simulink model "rfi_detection"  (R2013b)
settings: Solver=ode45  StartTime=0.0  StopTime=10.0  RelTol=1e-3
undefined symbols (not defined in the file or in its folder): calan_lib, comp_addsub
libraries: xbsIndex_r4 x2633, casper_library_misc x66, dspsigops x32, simulink x4, casper_library_delays x4, xps_library x2
(part 1 of 22)
settings Model: Creator=root  LastModifiedBy=root
settings DebuggingCC: StateNameClashWarn=warning

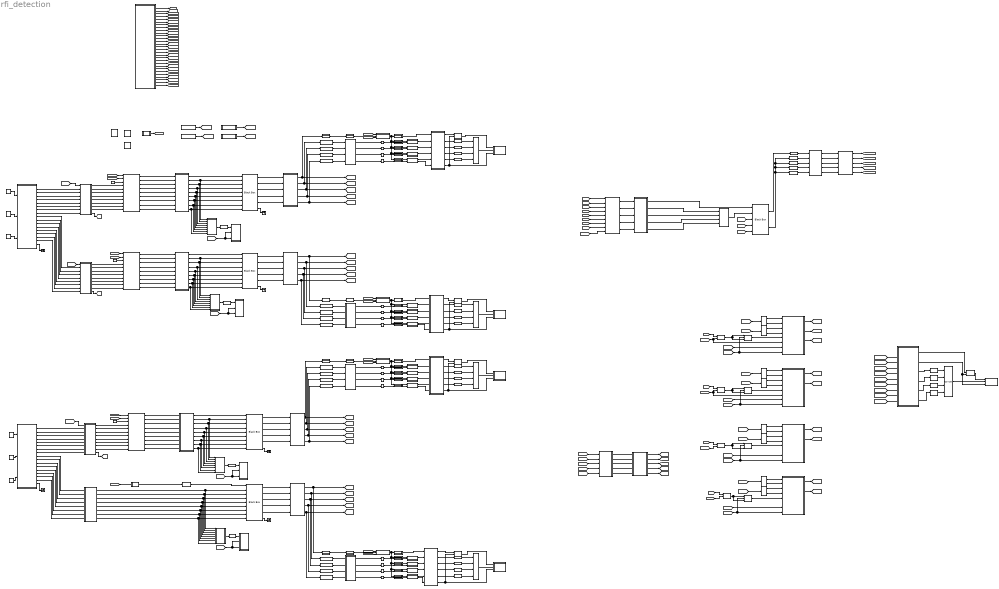
== system rfi_detection ==
  note: TODO!!!
  note: check if we could
      | hardcode the gain
  note: To catch the prog delay
  " System Generator" : xbsIndex_r4/ System Generator  Tag=genX  xilinxfamily=virtex6  part=xc6vsx475t  speed=-1  package=ff1759  synthesis_tool=XST  clock_wrapper=Clock Enables  directory=./arte/sysgen  proj_type=Project Navigator  Synth_file=XST Defaults  Impl_file=ISE Defaults  testbench=off  simulink_period=1  sysclk_period=6.6667  dcm_input_clock_period=100  incr_netlist=off  trim_vbits=Everywhere in SubSystem  dbl_ovrd=According to Block Masks  core_generation=According to Block Masks  run_coregen=off  deprecated_control=off  eval_field=0  block_type=sysgen
  Band-Limited White Noise{,1..3} (4 alike) : simulink/Sources/Band-Limited White Noise  Cov=[0.1]  Ts=0.1  seed=[23341]
  Black Box{1..3,6} (4 alike) : xbsIndex_r4/Black Box  init_code=pfb_fft_8in_2048ch_config  sim_method=Inactive  verbose=off  block_type=blackbox2
  Black Box5 : xbsIndex_r4/Black Box  init_code=fft_channel_flag_top_config  sim_method=Inactive  verbose=off  block_type=blackbox2
  Concat{,1..3,11} (5 alike) : xbsIndex_r4/Concat  num_inputs=4  dbl_ovrd=off  block_type=concat
  Constant11 : xbsIndex_r4/Constant  const=1  gui_display_data_type=Boolean  arith_type=Boolean  n_bits=16  bin_pt=14  preci_type=Single  exp_width=8  frac_width=24  explicit_period=on  period=1  equ=P=C  opselect=C  inp2=PCIN>>17  opr=+  inp1=P  carry=CIN  dbl_ovrd=off  block_type=constant
  Constant13 : Constant
  Constant2 : Constant
  Constant8 : xbsIndex_r4/Constant  const=1  gui_display_data_type=Boolean  arith_type=Boolean  n_bits=16  bin_pt=14  preci_type=Single  exp_width=8  frac_width=24  explicit_period=on  period=1  equ=P=C  opselect=C  inp2=PCIN>>17  opr=+  inp1=P  carry=CIN  dbl_ovrd=off  block_type=constant
  Constant9 : xbsIndex_r4/Constant  const=1  gui_display_data_type=Boolean  arith_type=Boolean  n_bits=16  bin_pt=14  preci_type=Single  exp_width=8  frac_width=24  explicit_period=on  period=1  equ=P=C  opselect=C  inp2=PCIN>>17  opr=+  inp1=P  carry=CIN  dbl_ovrd=off  block_type=constant
  Convert5 : xbsIndex_r4/Convert  gui_display_data_type=Boolean  arith_type=Boolean  n_bits=3  bin_pt=0  float_type=Single  exp_bits=8  fraction_bits=24  quantization=Truncate  overflow=Wrap  en=off  latency=0  dbl_ovrd=off  pipeline=off  block_type=convert
      settings: block_version=11.4
  Counter{1..4,10} (5 alike) : xbsIndex_r4/Counter  cnt_type=Free Running  cnt_to=Inf  operation=Up  start_count=0  cnt_by_val=1  arith_type=Unsigned  n_bits=9  bin_pt=0  load_pin=off  rst=on  en=on  explicit_period=on  period=1  dbl_ovrd=off  use_behavioral_HDL=off  implementation=Fabric  block_type=counter
  Delay{1,7..10,32,34..36,43,45..47,50..52} (16 alike) : xbsIndex_r4/Delay  rst=off  infoeditControl=Selection of Reset will increase slice count due to use of real FFs and instead of SRLs  en=off  latency=1  dbl_ovrd=off  reg_retiming=off  block_type=delay
  Logical{,1..3} (4 alike) : xbsIndex_r4/Logical  logical_function=AND  inputs=2  en=off  latency=0  precision=Full  arith_type=Unsigned  n_bits=16  bin_pt=0  align_bp=on  dbl_ovrd=off  block_type=logical
  Register{,1..3} (4 alike) : xbsIndex_r4/Register  init=0  rst=on  en=on  dbl_ovrd=off  block_type=register
  Reinterpret{1..12,21..26,28,31} (20 alike) : xbsIndex_r4/Reinterpret  force_arith_type=on  arith_type=Unsigned  force_bin_pt=on  bin_pt=0  block_type=reinterpret
  Slice1 : xbsIndex_r4/Slice  nbits=36  boolean_output=off  mode=Lower Bit Location + Width  bit1=0  base1=MSB of Input  bit0=72  base0=LSB of Input  dbl_ovrd=off  block_type=slice
  Slice2 : xbsIndex_r4/Slice  nbits=36  boolean_output=off  mode=Lower Bit Location + Width  bit1=0  base1=MSB of Input  bit0=108  base0=LSB of Input  dbl_ovrd=off  block_type=slice
  Slice3 : xbsIndex_r4/Slice  nbits=36  boolean_output=off  mode=Lower Bit Location + Width  bit1=0  base1=MSB of Input  bit0=0  base0=LSB of Input  dbl_ovrd=off  block_type=slice
  Slice5 : xbsIndex_r4/Slice  nbits=36  boolean_output=off  mode=Lower Bit Location + Width  bit1=0  base1=MSB of Input  bit0=36  base0=LSB of Input  dbl_ovrd=off  block_type=slice
  Subsystem : Subsystem
  Terminator{,1..2,4..5,18} (6 alike) : Terminator
  XSG_core_config : xps_library/XSG_core_config  Tag=xps:xsg  hw_sys=ROACH2:sx475t  clk_src=adc0_clk  ROACH_clk_src=sys_clk  ROACH2_clk_src=adc0_clk  MKDIG_clk_src=sys_clk  clk_rate=150  sample_period=1  synthesis_tool=XST
  acc_cntrl0 : Subsystem  mask{chan_bits=9}
      mask prompts: chan_bits "Number of Channels (2^?)"
  acc_cntrl1 : Subsystem  mask{chan_bits=9}
      mask prompts: chan_bits "Number of Channels (2^?)"
  acc_cntrl2 : Subsystem  mask{chan_bits=9}
      mask prompts: chan_bits "Number of Channels (2^?)"
  acc_cntrl3 : Subsystem  mask{chan_bits=9}
      mask prompts: chan_bits "Number of Channels (2^?)"
  acc_len : Subsystem  Tag=xps:sw_reg  AncestorBlock=xps_library/software_register  mask(swreg){io_dir=From Processor, io_delay=0, sample_period=1, names=reg, bitwidths=32, bin_pts=0, arith_types=0, sim_port=on, show_format=on}
      mask prompts: io_dir "I/O direction"; io_delay "I/O delay"; sample_period "Sample period"; names "Bitfield names [msb...lsb]"; bitwidths "Bitfield widths"; bin_pts "Bitfield binary pts"; arith_types "Bitfield types, ufix=0, fix=1, bool=2"; sim_port "Provide sim input/output?"; show_format "Print format string?"
      mask help: A 32-bit software-accessible register. Can be divided into bitfields of varying widths and types using the fields in the block mask.
      mask init:
      | try
      |     swreg_init(gcb)
      | catch ex
      |     disp(sprintf('%s: %s', gcb, ex.message))
      |     errordlg(ex.message)
      | end
      settings: AttributesFormatString=1input:uf32.0 = 32 bits
      mask TypeOptions io_dir: To Processor | From Processor
      mask Callback io_dir:
      | mask_enables = get_param(gcb, 'MaskEnables');
      | mask_names = get_param(gcb, 'MaskNames');
      | if strcmp(get_param(gcb, 'io_dir'), 'To Processor'),
      |     mask_enables{ismember(mask_names, 'sample_period')} = 'off';
      | else
      |     mask_enables{ismember(mask_names, 'sample_period')} = 'on';
      | end
      | set_param(gcb, 'MaskEnables', mask_enables);
  adcsnap0 : Subsystem  Tag=casper:snapshot  AncestorBlock=casper_library_scopes/snapshot  mask(snapshot){storage=bram, dram_dimm=1, dram_clock=200, nsamples=10, data_width=64, offset=on, circap=off, value=off, use_dsp48=off}
      mask prompts: storage "Storage medium"; dram_dimm "DRAM dimm"; dram_clock "DRAM clock rate"; nsamples "Number of Samples (2^?)"; data_width "Data width"; offset "Start delay support"; circap "Circular capture support"; value "Extra value capture support"; use_dsp48 "Use DSP48s to implement counters"
      mask help:
      | Standard snap block, but with the following optional extras;
      |  1) Optionally delay the fabric trigger by a user-specified number of valids.
      |  2) Capture continuously after a trigger until a stop pulse is received. Data is captured into BRAM continuously, with old data being overwritten until a stop command is received. Then stop capturing when memory is filled. This enables you to get some data before and some data after the stop pulse. Use the 'tr_en_cnt' register to determine where you are in your vector. 'Addr' register's MSb now indicates 'busy capturing'.
      |  3) Optionally capture a value on an input port to a register at the same time as the first data sample.
      |  4) Implement counters using DSP48Es to save resources.
      mask init:
      | snapshot_init(gcb, ...
      |     'storage', storage, ...
      |     'dram_dimm', dram_dimm, ...
      |     'dram_clock', dram_clock, ...
      |     'nsamples', nsamples, ...
      |     'data_width', data_width, ...
      |     'offset', offset, ...
      |     'circap', circap, ...
      |     'value', value, ...
      |     'use_dsp48', use_dsp48);
      mask TypeOptions storage: bram | dram
      mask Callback storage: snapshot_callback();
      mask TypeOptions dram_dimm: 1 | 2 | 3 | 4
      mask TypeOptions dram_clock: 200 | 250 | 266 | 300 | 333
      mask TypeOptions data_width: 8 | 16 | 32 | 64 | 128
  adcsnap1 : Subsystem  Tag=casper:snapshot  AncestorBlock=casper_library_scopes/snapshot  mask(snapshot){storage=bram, dram_dimm=1, dram_clock=200, nsamples=10, data_width=64, offset=on, circap=off, value=off, use_dsp48=off}
      mask prompts: storage "Storage medium"; dram_dimm "DRAM dimm"; dram_clock "DRAM clock rate"; nsamples "Number of Samples (2^?)"; data_width "Data width"; offset "Start delay support"; circap "Circular capture support"; value "Extra value capture support"; use_dsp48 "Use DSP48s to implement counters"
      mask help:
      | Standard snap block, but with the following optional extras;
      |  1) Optionally delay the fabric trigger by a user-specified number of valids.
      |  2) Capture continuously after a trigger until a stop pulse is received. Data is captured into BRAM continuously, with old data being overwritten until a stop command is received. Then stop capturing when memory is filled. This enables you to get some data before and some data after the stop pulse. Use the 'tr_en_cnt' register to determine where you are in your vector. 'Addr' register's MSb now indicates 'busy capturing'.
      |  3) Optionally capture a value on an input port to a register at the same time as the first data sample.
      |  4) Implement counters using DSP48Es to save resources.
      mask init: same as rfi_detection/adcsnap0
      mask TypeOptions storage: bram | dram
      mask Callback storage: snapshot_callback();
      mask TypeOptions dram_dimm: 1 | 2 | 3 | 4
      mask TypeOptions dram_clock: 200 | 250 | 266 | 300 | 333
      mask TypeOptions data_width: 8 | 16 | 32 | 64 | 128
  adcsnap2 : Subsystem  Tag=casper:snapshot  AncestorBlock=casper_library_scopes/snapshot  mask(snapshot){storage=bram, dram_dimm=1, dram_clock=200, nsamples=10, data_width=64, offset=on, circap=off, value=off, use_dsp48=off}
      mask prompts: storage "Storage medium"; dram_dimm "DRAM dimm"; dram_clock "DRAM clock rate"; nsamples "Number of Samples (2^?)"; data_width "Data width"; offset "Start delay support"; circap "Circular capture support"; value "Extra value capture support"; use_dsp48 "Use DSP48s to implement counters"
      mask help:
      | Standard snap block, but with the following optional extras;
      |  1) Optionally delay the fabric trigger by a user-specified number of valids.
      |  2) Capture continuously after a trigger until a stop pulse is received. Data is captured into BRAM continuously, with old data being overwritten until a stop command is received. Then stop capturing when memory is filled. This enables you to get some data before and some data after the stop pulse. Use the 'tr_en_cnt' register to determine where you are in your vector. 'Addr' register's MSb now indicates 'busy capturing'.
      |  3) Optionally capture a value on an input port to a register at the same time as the first data sample.
      |  4) Implement counters using DSP48Es to save resources.
      mask init: same as rfi_detection/adcsnap0
      mask TypeOptions storage: bram | dram
      mask Callback storage: snapshot_callback();
      mask TypeOptions dram_dimm: 1 | 2 | 3 | 4
      mask TypeOptions dram_clock: 200 | 250 | 266 | 300 | 333
      mask TypeOptions data_width: 8 | 16 | 32 | 64 | 128
  adcsnap3 : Subsystem  Tag=casper:snapshot  AncestorBlock=casper_library_scopes/snapshot  mask(snapshot){storage=bram, dram_dimm=1, dram_clock=200, nsamples=10, data_width=64, offset=on, circap=off, value=off, use_dsp48=off}
      mask prompts: storage "Storage medium"; dram_dimm "DRAM dimm"; dram_clock "DRAM clock rate"; nsamples "Number of Samples (2^?)"; data_width "Data width"; offset "Start delay support"; circap "Circular capture support"; value "Extra value capture support"; use_dsp48 "Use DSP48s to implement counters"
      mask help:
      | Standard snap block, but with the following optional extras;
      |  1) Optionally delay the fabric trigger by a user-specified number of valids.
      |  2) Capture continuously after a trigger until a stop pulse is received. Data is captured into BRAM continuously, with old data being overwritten until a stop command is received. Then stop capturing when memory is filled. This enables you to get some data before and some data after the stop pulse. Use the 'tr_en_cnt' register to determine where you are in your vector. 'Addr' register's MSb now indicates 'busy capturing'.
      |  3) Optionally capture a value on an input port to a register at the same time as the first data sample.
      |  4) Implement counters using DSP48Es to save resources.
      mask init: same as rfi_detection/adcsnap0
      mask TypeOptions storage: bram | dram
      mask Callback storage: snapshot_callback();
      mask TypeOptions dram_dimm: 1 | 2 | 3 | 4
      mask TypeOptions dram_clock: 200 | 250 | 266 | 300 | 333
      mask TypeOptions data_width: 8 | 16 | 32 | 64 | 128
  antenna_0 : Subsystem  Tag=xps:bram  AncestorBlock=xps_library/Shared_BRAM  mask{arith_type=Unsigned, addr_width=9, data_width=128, reg_prim_output=off, reg_core_output=off, optimization=Minimum_Area, data_bin_pt=0, init_vals=[0:2^10-1], sample_rate=1}
      mask prompts: arith_type "Output Data Type"; addr_width "Address width"; data_width "Data Width"; reg_prim_output "Register Primitive Output"; reg_core_output "Register Core Output"; data_bin_pt "Data Binary Point"; init_vals "Initial values (simulation only)"; sample_rate "Sample rate"
      mask init:
      | shared_bram_mask;
      mask TypeOptions arith_type: Unsigned | Signed  (2's comp)
      mask TypeOptions data_width: 8 | 16 | 32 | 64 | 128
      mask TypeOptions optimization: Minimum_Area | Low_Power
  antenna_1 : Subsystem  Tag=xps:bram  AncestorBlock=xps_library/Shared_BRAM  mask{arith_type=Unsigned, addr_width=9, data_width=128, reg_prim_output=off, reg_core_output=off, optimization=Minimum_Area, data_bin_pt=0, init_vals=[0:2^10-1], sample_rate=1}
      mask prompts: arith_type "Output Data Type"; addr_width "Address width"; data_width "Data Width"; reg_prim_output "Register Primitive Output"; reg_core_output "Register Core Output"; data_bin_pt "Data Binary Point"; init_vals "Initial values (simulation only)"; sample_rate "Sample rate"
      mask init:
      | shared_bram_mask;
      mask TypeOptions arith_type: Unsigned | Signed  (2's comp)
      mask TypeOptions data_width: 8 | 16 | 32 | 64 | 128
      mask TypeOptions optimization: Minimum_Area | Low_Power
  antenna_2 : Subsystem  Tag=xps:bram  AncestorBlock=xps_library/Shared_BRAM  mask{arith_type=Unsigned, addr_width=9, data_width=128, reg_prim_output=off, reg_core_output=off, optimization=Minimum_Area, data_bin_pt=0, init_vals=[0:2^10-1], sample_rate=1}
      mask prompts: arith_type "Output Data Type"; addr_width "Address width"; data_width "Data Width"; reg_prim_output "Register Primitive Output"; reg_core_output "Register Core Output"; data_bin_pt "Data Binary Point"; init_vals "Initial values (simulation only)"; sample_rate "Sample rate"
      mask init:
      | shared_bram_mask;
      mask TypeOptions arith_type: Unsigned | Signed  (2's comp)
      mask TypeOptions data_width: 8 | 16 | 32 | 64 | 128
      mask TypeOptions optimization: Minimum_Area | Low_Power
  antenna_3 : Subsystem  Tag=xps:bram  AncestorBlock=xps_library/Shared_BRAM  mask{arith_type=Unsigned, addr_width=9, data_width=128, reg_prim_output=off, reg_core_output=off, optimization=Minimum_Area, data_bin_pt=0, init_vals=[0:2^10-1], sample_rate=1}
      mask prompts: arith_type "Output Data Type"; addr_width "Address width"; data_width "Data Width"; reg_prim_output "Register Primitive Output"; reg_core_output "Register Core Output"; data_bin_pt "Data Binary Point"; init_vals "Initial values (simulation only)"; sample_rate "Sample rate"
      mask init:
      | shared_bram_mask;
      mask TypeOptions arith_type: Unsigned | Signed  (2's comp)
      mask TypeOptions data_width: 8 | 16 | 32 | 64 | 128
      mask TypeOptions optimization: Minimum_Area | Low_Power
  asiaa_adc5g0 : Subsystem  Tag=xps:adc5g  AncestorBlock=xps_library/ADCs/asiaa_adc5g  mask(adc5g){input_mode=Two-channel -- A&C, adc_brd=ZDOK 0, demux=1:1, adc_bit_width=8, adc_clk_rate=1200, using_ctrl=on, test_ramp=off}
      mask prompts: input_mode "Input mode:"; adc_brd "ADC Board"; demux "Internal demux"; adc_bit_width "ADC Resolution (bits):"; adc_clk_rate "ADC Clock Rate (MHz):"; using_ctrl "use control"; test_ramp "start in test ramp mode"
      mask help:
      | Interface for the ASIAA 5 GSps ADC. Supports interleaving all four
      | cores using either input A or C, or interleaving two-cores each for
      | A and C. The hardware itself comes in two versions:
      |
      | DMUX 1:2 -- 4-bit samples, 4 parallel streams
      | DMUX 1:1 -- 8-bit samples, 2 parallel streams
      |
      | In either configuration this block will output 8 parallel streams
      | but the underlying interface, and the bitwidth of the samples,
      | will be different.
      mask init:
      | adc5g_init(gcb,...
      |     'input_mode', input_mode,...
      |     'demux', demux,...
      |     'adc_clk_rate', adc_clk_rate,...
      |     'adc_bit_width', adc_bit_width,...
      |     'adc_brd', adc_brd,...
      |     'using_ctrl', using_ctrl,...
      |     'test_ramp', test_ramp);
      mask TypeOptions input_mode: One-channel -- A | One-channel -- C | Two-channel -- A&C
      mask TypeOptions adc_brd: ZDOK 0 | ZDOK 1
      mask TypeOptions demux: 1:1 | 1:2
      mask Callback demux:
      | demux = get_param(gcb,'demux');
      | if(strcmp(demux,'1:1')),
      |     set_param(gcb, 'adc_bit_width', '8')
      | elseif(strcmp(demux, '1:2')),
      |     set_param(gcb, 'adc_bit_width', '4');
      | else
      | end
  asiaa_adc5g1 : Subsystem  Tag=xps:adc5g  AncestorBlock=xps_library/ADCs/asiaa_adc5g  mask(adc5g){input_mode=Two-channel -- A&C, adc_brd=ZDOK 1, demux=1:1, adc_bit_width=8, adc_clk_rate=1200, using_ctrl=on, test_ramp=off}
      mask prompts: input_mode "Input mode:"; adc_brd "ADC Board"; demux "Internal demux"; adc_bit_width "ADC Resolution (bits):"; adc_clk_rate "ADC Clock Rate (MHz):"; using_ctrl "use control"; test_ramp "start in test ramp mode"
      mask help:
      | Interface for the ASIAA 5 GSps ADC. Supports interleaving all four
      | cores using either input A or C, or interleaving two-cores each for
      | A and C. The hardware itself comes in two versions:
      |
      | DMUX 1:2 -- 4-bit samples, 4 parallel streams
      | DMUX 1:1 -- 8-bit samples, 2 parallel streams
      |
      | In either configuration this block will output 8 parallel streams
      | but the underlying interface, and the bitwidth of the samples,
      | will be different.
      mask init: same as rfi_detection/asiaa_adc5g0
      mask TypeOptions input_mode: One-channel -- A | One-channel -- C | Two-channel -- A&C
      mask TypeOptions adc_brd: ZDOK 0 | ZDOK 1
      mask TypeOptions demux: 1:1 | 1:2
      mask Callback demux:
      | demux = get_param(gcb,'demux');
      | if(strcmp(demux,'1:1')),
      |     set_param(gcb, 'adc_bit_width', '8')
      | elseif(strcmp(demux, '1:2')),
      |     set_param(gcb, 'adc_bit_width', '4');
      | else
      | end
  beam_post_complex_add : Subsystem  mask{lat=3}
  beam_rfi_convert : Subsystem  mask{shift_val=9, conv_width=9, conv_point=8}
      mask prompts: shift_val "shift"; conv_width "convert width"; conv_point "convert point"
  beam_rfi_delay : Subsystem  mask{lat=3}
  bus_create : Subsystem  AncestorBlock=casper_library_flow_control/bus_create  mask(bus_create){inputNum=8}
      mask prompts: inputNum "Number of inputs:"
      mask init:
      | bus_create_init(gcb,...
      |     'inputNum', inputNum);
  bus_create1 : Subsystem  AncestorBlock=casper_library_flow_control/bus_create  mask(bus_create){inputNum=8}
      mask prompts: inputNum "Number of inputs:"
      mask init:
      | bus_create_init(gcb,...
      |     'inputNum', inputNum);
  bus_create2 : Subsystem  AncestorBlock=casper_library_flow_control/bus_create  mask(bus_create){inputNum=8}
      mask prompts: inputNum "Number of inputs:"
      mask init:
      | bus_create_init(gcb,...
      |     'inputNum', inputNum);
  bus_create3 : Subsystem  AncestorBlock=casper_library_flow_control/bus_create  mask(bus_create){inputNum=8}
      mask prompts: inputNum "Number of inputs:"
      mask init:
      | bus_create_init(gcb,...
      |     'inputNum', inputNum);
  c_to_ri{,1..7} (8 alike) : casper_library_misc/c_to_ri  n_bits=18  bin_pt=17
  cnt_rst : Subsystem  Tag=xps:sw_reg  AncestorBlock=xps_library/software_register  mask(swreg){io_dir=From Processor, io_delay=0, sample_period=1, names=reg, bitwidths=32, bin_pts=0, arith_types=2, sim_port=on, show_format=on}
      mask prompts: io_dir "I/O direction"; io_delay "I/O delay"; sample_period "Sample period"; names "Bitfield names [msb...lsb]"; bitwidths "Bitfield widths"; bin_pts "Bitfield binary pts"; arith_types "Bitfield types, ufix=0, fix=1, bool=2"; sim_port "Provide sim input/output?"; show_format "Print format string?"
      mask help: A 32-bit software-accessible register. Can be divided into bitfields of varying widths and types using the fields in the block mask.
      mask init:
      | try
      |     swreg_init(gcb)
      | catch ex
      |     disp(sprintf('%s: %s', gcb, ex.message))
      |     errordlg(ex.message)
      | end
      settings: AttributesFormatString=1input:b = 32 bits
      mask TypeOptions io_dir: To Processor | From Processor
      mask Callback io_dir:
      | mask_enables = get_param(gcb, 'MaskEnables');
      | mask_names = get_param(gcb, 'MaskNames');
      | if strcmp(get_param(gcb, 'io_dir'), 'To Processor'),
      |     mask_enables{ismember(mask_names, 'sample_period')} = 'off';
      | else
      |     mask_enables{ismember(mask_names, 'sample_period')} = 'on';
      | end
      | set_param(gcb, 'MaskEnables', mask_enables);
  complex_add : Subsystem
  concat_order : Subsystem
  control : Subsystem
  conv_bus1 : Subsystem
  conv_bus2 : Subsystem
  conv_bus4 : Subsystem
  delay_pre_pfb : xbsIndex_r4/Delay  rst=off  infoeditControl=Selection of Reset will increase slice count due to use of real FFs and instead of SRLs  en=off  latency=1  dbl_ovrd=off  reg_retiming=off  block_type=delay
  delay_wideband_prog0 : Subsystem  AncestorBlock=casper_library_delays/delay_wideband_prog  mask(delay_wideband_prog){max_delay=128, n_inputs_bits=3, bram_latency=2, bram_type=Dual Port, async=off}
      mask prompts: max_delay "Max Delay (Sample Clks)"; n_inputs_bits "Number of Simultaneous Inputs(2^?)"; bram_latency "BRAM Latency"; bram_type "Select type of BRAM"; async "asynchronous operation"
      mask init:
      | delay_wideband_prog_init(gcb,...
      |     'max_delay',max_delay,...
      |     'n_inputs_bits',n_inputs_bits,...
      |     'bram_latency',bram_latency,...
      |     'bram_type',bram_type, ...
      |     'async', async);
      mask TypeOptions bram_type: Single Port | Dual Port
  delay_wideband_prog1 : Subsystem  AncestorBlock=casper_library_delays/delay_wideband_prog  mask(delay_wideband_prog){max_delay=128, n_inputs_bits=3, bram_latency=2, bram_type=Dual Port, async=off}
      mask prompts: max_delay "Max Delay (Sample Clks)"; n_inputs_bits "Number of Simultaneous Inputs(2^?)"; bram_latency "BRAM Latency"; bram_type "Select type of BRAM"; async "asynchronous operation"
      mask init:
      | delay_wideband_prog_init(gcb,...
      |     'max_delay',max_delay,...
      |     'n_inputs_bits',n_inputs_bits,...
      |     'bram_latency',bram_latency,...
      |     'bram_type',bram_type, ...
      |     'async', async);
      mask TypeOptions bram_type: Single Port | Dual Port
  delay_wideband_prog2 : Subsystem  AncestorBlock=casper_library_delays/delay_wideband_prog  mask(delay_wideband_prog){max_delay=128, n_inputs_bits=3, bram_latency=2, bram_type=Dual Port, async=off}
      mask prompts: max_delay "Max Delay (Sample Clks)"; n_inputs_bits "Number of Simultaneous Inputs(2^?)"; bram_latency "BRAM Latency"; bram_type "Select type of BRAM"; async "asynchronous operation"
      mask init:
      | delay_wideband_prog_init(gcb,...
      |     'max_delay',max_delay,...
      |     'n_inputs_bits',n_inputs_bits,...
      |     'bram_latency',bram_latency,...
      |     'bram_type',bram_type, ...
      |     'async', async);
      mask TypeOptions bram_type: Single Port | Dual Port
  pcore : xps_library/pcore  Tag=xps:pcore  pcore_path=pfb_fft_8in_2048ch.ngc
  phase_calc : Subsystem  mask{din_width=18, din_point=8, scale_max_shift=0, scale_min_shift=0, pre_cordic_shift=0, pre_cordic_width=16, pre_cordic_point=6, cordic_iters=16}
      mask prompts: din_width "din width"; din_point "din point"; scale_max_shift "autoscale max shift"; scale_min_shift "autoscale min shift"; pre_cordic_shift "pre cordic shift"; pre_cordic_width "pre cordic width"; pre_cordic_point "pre cordic point"; cordic_iters "cordic iters"
  pipeline : Subsystem  AncestorBlock=casper_library_delays/pipeline  mask(pipeline){latency=6}
      mask help:
      | An explicitly laid-out delay line to avoid mapping to SRL16s
      | for use in pipelining to help achieve timing closure.
      mask init:
      | pipeline_init(gcb,'latency',latency);
      settings: AttributesFormatString=Latency = %<latency>
      mask Display:
      | port_label('input', 1, 'd');
      | port_label('output', 1, 'q');
      | disp(['Z^-', num2str(latency)]);
  pipeline102 : Subsystem  AncestorBlock=casper_library_delays/pipeline  mask(pipeline){latency=1}
      mask help:
      | An explicitly laid-out delay line to avoid mapping to SRL16s
      | for use in pipelining to help achieve timing closure.
      mask init:
      | pipeline_init(gcb,'latency',latency);
      settings: AttributesFormatString=Latency = %<latency>
      mask Display:
      | port_label('input', 1, 'd');
      | port_label('output', 1, 'q');
      | disp(['Z^-', num2str(latency)]);
  pipeline103 : Subsystem  AncestorBlock=casper_library_delays/pipeline  mask(pipeline){latency=5}
      mask help:
      | An explicitly laid-out delay line to avoid mapping to SRL16s
      | for use in pipelining to help achieve timing closure.
      mask init:
      | pipeline_init(gcb,'latency',latency);
      settings: AttributesFormatString=Latency = %<latency>
      mask Display:
      | port_label('input', 1, 'd');
      | port_label('output', 1, 'q');
      | disp(['Z^-', num2str(latency)]);
  pipeline104 : Subsystem  AncestorBlock=casper_library_delays/pipeline  mask(pipeline){latency=1}
      mask help:
      | An explicitly laid-out delay line to avoid mapping to SRL16s
      | for use in pipelining to help achieve timing closure.
      mask init:
      | pipeline_init(gcb,'latency',latency);
      settings: AttributesFormatString=Latency = %<latency>
      mask Display:
      | port_label('input', 1, 'd');
      | port_label('output', 1, 'q');
      | disp(['Z^-', num2str(latency)]);
  pipeline107 : Subsystem  AncestorBlock=casper_library_delays/pipeline  mask(pipeline){latency=1}
      mask help:
      | An explicitly laid-out delay line to avoid mapping to SRL16s
      | for use in pipelining to help achieve timing closure.
      mask init:
      | pipeline_init(gcb,'latency',latency);
      settings: AttributesFormatString=Latency = %<latency>
      mask Display:
      | port_label('input', 1, 'd');
      | port_label('output', 1, 'q');
      | disp(['Z^-', num2str(latency)]);
  pipeline108 : Subsystem  AncestorBlock=casper_library_delays/pipeline  mask(pipeline){latency=1}
      mask help:
      | An explicitly laid-out delay line to avoid mapping to SRL16s
      | for use in pipelining to help achieve timing closure.
      mask init:
      | pipeline_init(gcb,'latency',latency);
      settings: AttributesFormatString=Latency = %<latency>
      mask Display:
      | port_label('input', 1, 'd');
      | port_label('output', 1, 'q');
      | disp(['Z^-', num2str(latency)]);
  pipeline109 : Subsystem  AncestorBlock=casper_library_delays/pipeline  mask(pipeline){latency=1}
      mask help:
      | An explicitly laid-out delay line to avoid mapping to SRL16s
      | for use in pipelining to help achieve timing closure.
      mask init:
      | pipeline_init(gcb,'latency',latency);
      settings: AttributesFormatString=Latency = %<latency>
      mask Display:
      | port_label('input', 1, 'd');
      | port_label('output', 1, 'q');
      | disp(['Z^-', num2str(latency)]);
  pipeline112 : Subsystem  AncestorBlock=casper_library_delays/pipeline  mask(pipeline){latency=1}
      mask help:
      | An explicitly laid-out delay line to avoid mapping to SRL16s
      | for use in pipelining to help achieve timing closure.
      mask init:
      | pipeline_init(gcb,'latency',latency);
      settings: AttributesFormatString=Latency = %<latency>
      mask Display:
      | port_label('input', 1, 'd');
      | port_label('output', 1, 'q');
      | disp(['Z^-', num2str(latency)]);
  pipeline113 : Subsystem  AncestorBlock=casper_library_delays/pipeline  mask(pipeline){latency=1}
      mask help:
      | An explicitly laid-out delay line to avoid mapping to SRL16s
      | for use in pipelining to help achieve timing closure.
      mask init:
      | pipeline_init(gcb,'latency',latency);
      settings: AttributesFormatString=Latency = %<latency>
      mask Display:
      | port_label('input', 1, 'd');
      | port_label('output', 1, 'q');
      | disp(['Z^-', num2str(latency)]);
  pipeline116 : Subsystem  AncestorBlock=casper_library_delays/pipeline  mask(pipeline){latency=1}
      mask help:
      | An explicitly laid-out delay line to avoid mapping to SRL16s
      | for use in pipelining to help achieve timing closure.
      mask init:
      | pipeline_init(gcb,'latency',latency);
      settings: AttributesFormatString=Latency = %<latency>
      mask Display:
      | port_label('input', 1, 'd');
      | port_label('output', 1, 'q');
      | disp(['Z^-', num2str(latency)]);
  pipeline117 : Subsystem  AncestorBlock=casper_library_delays/pipeline  mask(pipeline){latency=1}
      mask help:
      | An explicitly laid-out delay line to avoid mapping to SRL16s
      | for use in pipelining to help achieve timing closure.
      mask init:
      | pipeline_init(gcb,'latency',latency);
      settings: AttributesFormatString=Latency = %<latency>
      mask Display:
      | port_label('input', 1, 'd');
      | port_label('output', 1, 'q');
      | disp(['Z^-', num2str(latency)]);
  pipeline120 : Subsystem  AncestorBlock=casper_library_delays/pipeline  mask(pipeline){latency=1}
      mask help:
      | An explicitly laid-out delay line to avoid mapping to SRL16s
      | for use in pipelining to help achieve timing closure.
      mask init:
      | pipeline_init(gcb,'latency',latency);
      settings: AttributesFormatString=Latency = %<latency>
      mask Display:
      | port_label('input', 1, 'd');
      | port_label('output', 1, 'q');
      | disp(['Z^-', num2str(latency)]);
  pipeline122 : Subsystem  AncestorBlock=casper_library_delays/pipeline  mask(pipeline){latency=5}
      mask help:
      | An explicitly laid-out delay line to avoid mapping to SRL16s
      | for use in pipelining to help achieve timing closure.
      mask init:
      | pipeline_init(gcb,'latency',latency);
      settings: AttributesFormatString=Latency = %<latency>
      mask Display:
      | port_label('input', 1, 'd');
      | port_label('output', 1, 'q');
      | disp(['Z^-', num2str(latency)]);
  pipeline123 : Subsystem  AncestorBlock=casper_library_delays/pipeline  mask(pipeline){latency=1}
      mask help:
      | An explicitly laid-out delay line to avoid mapping to SRL16s
      | for use in pipelining to help achieve timing closure.
      mask init:
      | pipeline_init(gcb,'latency',latency);
      settings: AttributesFormatString=Latency = %<latency>
      mask Display:
      | port_label('input', 1, 'd');
      | port_label('output', 1, 'q');
      | disp(['Z^-', num2str(latency)]);
  pipeline127 : Subsystem  AncestorBlock=casper_library_delays/pipeline  mask(pipeline){latency=2}
      mask help:
      | An explicitly laid-out delay line to avoid mapping to SRL16s
      | for use in pipelining to help achieve timing closure.
      mask init:
      | pipeline_init(gcb,'latency',latency);
      settings: AttributesFormatString=Latency = %<latency>
      mask Display:
      | port_label('input', 1, 'd');
      | port_label('output', 1, 'q');
      | disp(['Z^-', num2str(latency)]);
  pipeline128 : Subsystem  AncestorBlock=casper_library_delays/pipeline  mask(pipeline){latency=2}
      mask help:
      | An explicitly laid-out delay line to avoid mapping to SRL16s
      | for use in pipelining to help achieve timing closure.
      mask init:
      | pipeline_init(gcb,'latency',latency);
      settings: AttributesFormatString=Latency = %<latency>
      mask Display:
      | port_label('input', 1, 'd');
      | port_label('output', 1, 'q');
      | disp(['Z^-', num2str(latency)]);
  pipeline129 : Subsystem  AncestorBlock=casper_library_delays/pipeline  mask(pipeline){latency=2}
      mask help:
      | An explicitly laid-out delay line to avoid mapping to SRL16s
      | for use in pipelining to help achieve timing closure.
      mask init:
      | pipeline_init(gcb,'latency',latency);
      settings: AttributesFormatString=Latency = %<latency>
      mask Display:
      | port_label('input', 1, 'd');
      | port_label('output', 1, 'q');
      | disp(['Z^-', num2str(latency)]);
  pipeline130 : Subsystem  AncestorBlock=casper_library_delays/pipeline  mask(pipeline){latency=2}
      mask help:
      | An explicitly laid-out delay line to avoid mapping to SRL16s
      | for use in pipelining to help achieve timing closure.
      mask init:
      | pipeline_init(gcb,'latency',latency);
      settings: AttributesFormatString=Latency = %<latency>
      mask Display:
      | port_label('input', 1, 'd');
      | port_label('output', 1, 'q');
      | disp(['Z^-', num2str(latency)]);
  pipeline{4,6,44,276} (4 alike) : casper_library_delays/pipeline  latency=3
      settings: AttributesFormatString=Latency = %<latency>
  pipeline49 : Subsystem  AncestorBlock=casper_library_delays/pipeline  mask(pipeline){latency=1}
      mask help:
      | An explicitly laid-out delay line to avoid mapping to SRL16s
      | for use in pipelining to help achieve timing closure.
      mask init:
      | pipeline_init(gcb,'latency',latency);
      settings: AttributesFormatString=Latency = %<latency>
      mask Display:
      | port_label('input', 1, 'd');
      | port_label('output', 1, 'q');
      | disp(['Z^-', num2str(latency)]);
  pipeline50 : Subsystem  AncestorBlock=casper_library_delays/pipeline  mask(pipeline){latency=1}
      mask help:
      | An explicitly laid-out delay line to avoid mapping to SRL16s
      | for use in pipelining to help achieve timing closure.
      mask init:
      | pipeline_init(gcb,'latency',latency);
      settings: AttributesFormatString=Latency = %<latency>
      mask Display:
      | port_label('input', 1, 'd');
      | port_label('output', 1, 'q');
      | disp(['Z^-', num2str(latency)]);
  pipeline52 : Subsystem  AncestorBlock=casper_library_delays/pipeline  mask(pipeline){latency=1}
      mask help:
      | An explicitly laid-out delay line to avoid mapping to SRL16s
      | for use in pipelining to help achieve timing closure.
      mask init:
      | pipeline_init(gcb,'latency',latency);
      settings: AttributesFormatString=Latency = %<latency>
      mask Display:
      | port_label('input', 1, 'd');
      | port_label('output', 1, 'q');
      | disp(['Z^-', num2str(latency)]);
  pipeline55 : Subsystem  AncestorBlock=casper_library_delays/pipeline  mask(pipeline){latency=1}
      mask help:
      | An explicitly laid-out delay line to avoid mapping to SRL16s
      | for use in pipelining to help achieve timing closure.
      mask init:
      | pipeline_init(gcb,'latency',latency);
      settings: AttributesFormatString=Latency = %<latency>
      mask Display:
      | port_label('input', 1, 'd');
      | port_label('output', 1, 'q');
      | disp(['Z^-', num2str(latency)]);
  pipeline58 : Subsystem  AncestorBlock=casper_library_delays/pipeline  mask(pipeline){latency=1}
      mask help:
      | An explicitly laid-out delay line to avoid mapping to SRL16s
      | for use in pipelining to help achieve timing closure.
      mask init:
      | pipeline_init(gcb,'latency',latency);
      settings: AttributesFormatString=Latency = %<latency>
      mask Display:
      | port_label('input', 1, 'd');
      | port_label('output', 1, 'q');
      | disp(['Z^-', num2str(latency)]);
  pipeline59 : Subsystem  AncestorBlock=casper_library_delays/pipeline  mask(pipeline){latency=1}
      mask help:
      | An explicitly laid-out delay line to avoid mapping to SRL16s
      | for use in pipelining to help achieve timing closure.
      mask init:
      | pipeline_init(gcb,'latency',latency);
      settings: AttributesFormatString=Latency = %<latency>
      mask Display:
      | port_label('input', 1, 'd');
      | port_label('output', 1, 'q');
      | disp(['Z^-', num2str(latency)]);
  pipeline60 : Subsystem  AncestorBlock=casper_library_delays/pipeline  mask(pipeline){latency=1}
      mask help:
      | An explicitly laid-out delay line to avoid mapping to SRL16s
      | for use in pipelining to help achieve timing closure.
      mask init:
      | pipeline_init(gcb,'latency',latency);
      settings: AttributesFormatString=Latency = %<latency>
      mask Display:
      | port_label('input', 1, 'd');
      | port_label('output', 1, 'q');
      | disp(['Z^-', num2str(latency)]);
  pipeline63 : Subsystem  AncestorBlock=casper_library_delays/pipeline  mask(pipeline){latency=1}
      mask help:
      | An explicitly laid-out delay line to avoid mapping to SRL16s
      | for use in pipelining to help achieve timing closure.
      mask init:
      | pipeline_init(gcb,'latency',latency);
      settings: AttributesFormatString=Latency = %<latency>
      mask Display:
      | port_label('input', 1, 'd');
      | port_label('output', 1, 'q');
      | disp(['Z^-', num2str(latency)]);
  pipeline64 : Subsystem  AncestorBlock=casper_library_delays/pipeline  mask(pipeline){latency=1}
      mask help:
      | An explicitly laid-out delay line to avoid mapping to SRL16s
      | for use in pipelining to help achieve timing closure.
      mask init:
      | pipeline_init(gcb,'latency',latency);
      settings: AttributesFormatString=Latency = %<latency>
      mask Display:
      | port_label('input', 1, 'd');
      | port_label('output', 1, 'q');
      | disp(['Z^-', num2str(latency)]);
  pipeline67 : Subsystem  AncestorBlock=casper_library_delays/pipeline  mask(pipeline){latency=1}
      mask help:
      | An explicitly laid-out delay line to avoid mapping to SRL16s
      | for use in pipelining to help achieve timing closure.
      mask init:
      | pipeline_init(gcb,'latency',latency);
      settings: AttributesFormatString=Latency = %<latency>
      mask Display:
      | port_label('input', 1, 'd');
      | port_label('output', 1, 'q');
      | disp(['Z^-', num2str(latency)]);
  pipeline68 : Subsystem  AncestorBlock=casper_library_delays/pipeline  mask(pipeline){latency=1}
      mask help:
      | An explicitly laid-out delay line to avoid mapping to SRL16s
      | for use in pipelining to help achieve timing closure.
      mask init:
      | pipeline_init(gcb,'latency',latency);
      settings: AttributesFormatString=Latency = %<latency>
      mask Display:
      | port_label('input', 1, 'd');
      | port_label('output', 1, 'q');
      | disp(['Z^-', num2str(latency)]);
  pipeline71 : Subsystem  AncestorBlock=casper_library_delays/pipeline  mask(pipeline){latency=1}
      mask help:
      | An explicitly laid-out delay line to avoid mapping to SRL16s
      | for use in pipelining to help achieve timing closure.
      mask init:
      | pipeline_init(gcb,'latency',latency);
      settings: AttributesFormatString=Latency = %<latency>
      mask Display:
      | port_label('input', 1, 'd');
      | port_label('output', 1, 'q');
      | disp(['Z^-', num2str(latency)]);
  pipeline72 : Subsystem  AncestorBlock=casper_library_delays/pipeline  mask(pipeline){latency=5}
      mask help:
      | An explicitly laid-out delay line to avoid mapping to SRL16s
      | for use in pipelining to help achieve timing closure.
      mask init:
      | pipeline_init(gcb,'latency',latency);
      settings: AttributesFormatString=Latency = %<latency>
      mask Display:
      | port_label('input', 1, 'd');
      | port_label('output', 1, 'q');
      | disp(['Z^-', num2str(latency)]);
  pipeline73 : Subsystem  AncestorBlock=casper_library_delays/pipeline  mask(pipeline){latency=1}
      mask help:
      | An explicitly laid-out delay line to avoid mapping to SRL16s
      | for use in pipelining to help achieve timing closure.
      mask init:
      | pipeline_init(gcb,'latency',latency);
      settings: AttributesFormatString=Latency = %<latency>
      mask Display:
      | port_label('input', 1, 'd');
      | port_label('output', 1, 'q');
      | disp(['Z^-', num2str(latency)]);
  pipeline76 : Subsystem  AncestorBlock=casper_library_delays/pipeline  mask(pipeline){latency=1}
      mask help:
      | An explicitly laid-out delay line to avoid mapping to SRL16s
      | for use in pipelining to help achieve timing closure.
      mask init:
      | pipeline_init(gcb,'latency',latency);
      settings: AttributesFormatString=Latency = %<latency>
      mask Display:
      | port_label('input', 1, 'd');
      | port_label('output', 1, 'q');
      | disp(['Z^-', num2str(latency)]);
  pipeline77 : Subsystem  AncestorBlock=casper_library_delays/pipeline  mask(pipeline){latency=1}
      mask help:
      | An explicitly laid-out delay line to avoid mapping to SRL16s
      | for use in pipelining to help achieve timing closure.
      mask init:
      | pipeline_init(gcb,'latency',latency);
      settings: AttributesFormatString=Latency = %<latency>
      mask Display:
      | port_label('input', 1, 'd');
      | port_label('output', 1, 'q');
      | disp(['Z^-', num2str(latency)]);
  pipeline78 : Subsystem  AncestorBlock=casper_library_delays/pipeline  mask(pipeline){latency=1}
      mask help:
      | An explicitly laid-out delay line to avoid mapping to SRL16s
      | for use in pipelining to help achieve timing closure.
      mask init:
      | pipeline_init(gcb,'latency',latency);
      settings: AttributesFormatString=Latency = %<latency>
      mask Display:
      | port_label('input', 1, 'd');
      | port_label('output', 1, 'q');
      | disp(['Z^-', num2str(latency)]);
  pipeline81 : Subsystem  AncestorBlock=casper_library_delays/pipeline  mask(pipeline){latency=1}
      mask help:
      | An explicitly laid-out delay line to avoid mapping to SRL16s
      | for use in pipelining to help achieve timing closure.
      mask init:
      | pipeline_init(gcb,'latency',latency);
      settings: AttributesFormatString=Latency = %<latency>
      mask Display:
      | port_label('input', 1, 'd');
      | port_label('output', 1, 'q');
      | disp(['Z^-', num2str(latency)]);
  pipeline82 : Subsystem  AncestorBlock=casper_library_delays/pipeline  mask(pipeline){latency=1}
      mask help:
      | An explicitly laid-out delay line to avoid mapping to SRL16s
      | for use in pipelining to help achieve timing closure.
      mask init:
      | pipeline_init(gcb,'latency',latency);
      settings: AttributesFormatString=Latency = %<latency>
      mask Display:
      | port_label('input', 1, 'd');
      | port_label('output', 1, 'q');
      | disp(['Z^-', num2str(latency)]);
  pipeline85 : Subsystem  AncestorBlock=casper_library_delays/pipeline  mask(pipeline){latency=1}
      mask help:
      | An explicitly laid-out delay line to avoid mapping to SRL16s
      | for use in pipelining to help achieve timing closure.
      mask init:
      | pipeline_init(gcb,'latency',latency);
      settings: AttributesFormatString=Latency = %<latency>
      mask Display:
      | port_label('input', 1, 'd');
      | port_label('output', 1, 'q');
      | disp(['Z^-', num2str(latency)]);
  pipeline86 : Subsystem  AncestorBlock=casper_library_delays/pipeline  mask(pipeline){latency=1}
      mask help:
      | An explicitly laid-out delay line to avoid mapping to SRL16s
      | for use in pipelining to help achieve timing closure.
      mask init:
      | pipeline_init(gcb,'latency',latency);
      settings: AttributesFormatString=Latency = %<latency>
      mask Display:
      | port_label('input', 1, 'd');
      | port_label('output', 1, 'q');
      | disp(['Z^-', num2str(latency)]);
  pipeline89 : Subsystem  AncestorBlock=casper_library_delays/pipeline  mask(pipeline){latency=1}
      mask help:
      | An explicitly laid-out delay line to avoid mapping to SRL16s
      | for use in pipelining to help achieve timing closure.
      mask init:
      | pipeline_init(gcb,'latency',latency);
      settings: AttributesFormatString=Latency = %<latency>
      mask Display:
      | port_label('input', 1, 'd');
      | port_label('output', 1, 'q');
      | disp(['Z^-', num2str(latency)]);
  pipeline90 : Subsystem  AncestorBlock=casper_library_delays/pipeline  mask(pipeline){latency=5}
      mask help:
      | An explicitly laid-out delay line to avoid mapping to SRL16s
      | for use in pipelining to help achieve timing closure.
      mask init:
      | pipeline_init(gcb,'latency',latency);
      settings: AttributesFormatString=Latency = %<latency>
      mask Display:
      | port_label('input', 1, 'd');
      | port_label('output', 1, 'q');
      | disp(['Z^-', num2str(latency)]);
  pipeline91 : Subsystem  AncestorBlock=casper_library_delays/pipeline  mask(pipeline){latency=1}
      mask help:
      | An explicitly laid-out delay line to avoid mapping to SRL16s
      | for use in pipelining to help achieve timing closure.
      mask init:
      | pipeline_init(gcb,'latency',latency);
      settings: AttributesFormatString=Latency = %<latency>
      mask Display:
      | port_label('input', 1, 'd');
      | port_label('output', 1, 'q');
      | disp(['Z^-', num2str(latency)]);
  pipeline94 : Subsystem  AncestorBlock=casper_library_delays/pipeline  mask(pipeline){latency=1}
      mask help:
      | An explicitly laid-out delay line to avoid mapping to SRL16s
      | for use in pipelining to help achieve timing closure.
      mask init:
      | pipeline_init(gcb,'latency',latency);
      settings: AttributesFormatString=Latency = %<latency>
      mask Display:
      | port_label('input', 1, 'd');
      | port_label('output', 1, 'q');
      | disp(['Z^-', num2str(latency)]);
  pipeline97 : Subsystem  AncestorBlock=casper_library_delays/pipeline  mask(pipeline){latency=1}
      mask help:
      | An explicitly laid-out delay line to avoid mapping to SRL16s
      | for use in pipelining to help achieve timing closure.
      mask init:
      | pipeline_init(gcb,'latency',latency);
      settings: AttributesFormatString=Latency = %<latency>
      mask Display:
      | port_label('input', 1, 'd');
      | port_label('output', 1, 'q');
      | disp(['Z^-', num2str(latency)]);
  pipeline98 : Subsystem  AncestorBlock=casper_library_delays/pipeline  mask(pipeline){latency=1}
      mask help:
      | An explicitly laid-out delay line to avoid mapping to SRL16s
      | for use in pipelining to help achieve timing closure.
      mask init:
      | pipeline_init(gcb,'latency',latency);
      settings: AttributesFormatString=Latency = %<latency>
      mask Display:
      | port_label('input', 1, 'd');
      | port_label('output', 1, 'q');
      | disp(['Z^-', num2str(latency)]);
  post_fft_delay0 : Subsystem  mask{lat=3}
  post_fft_delay1 : Subsystem  mask{lat=3}
  post_fft_delay2 : Subsystem  mask{lat=3}
  post_fft_delay3 : Subsystem  mask{lat=3}
  power{1..16} (16 alike) : casper_library_misc/power  BitWidth=18  add_latency=2  mult_latency=3
  power_convert0 : Subsystem  mask{shift_val=13, conv_width=20, conv_point=19}
      mask prompts: shift_val "shift"; conv_width "convert width"; conv_point "convert point"
  power_convert1 : Subsystem  mask{shift_val=13, conv_width=20, conv_point=19}
      mask prompts: shift_val "shift"; conv_width "convert width"; conv_point "convert point"
  power_convert2 : Subsystem  mask{shift_val=13, conv_width=20, conv_point=19}
      mask prompts: shift_val "shift"; conv_width "convert width"; conv_point "convert point"
  power_convert3 : Subsystem  mask{shift_val=13, conv_width=20, conv_point=19}
      mask prompts: shift_val "shift"; conv_width "convert width"; conv_point "convert point"
  pre_bram_delay0 : Subsystem  mask{lat=2}
  pre_bram_delay1 : Subsystem  mask{lat=2}
  pre_bram_delay2 : Subsystem  mask{lat=2}
  pre_bram_delay3 : Subsystem  mask{lat=2}
  pre_pfb_delay1 : Subsystem  mask{lat=1}
  pre_pfb_delay2 : Subsystem  mask{lat=1}
  pre_pfb_delay3 : Subsystem  mask{lat=1}
  rfi_acc_len : Subsystem  Tag=xps:sw_reg  AncestorBlock=xps_library/software_register  mask(swreg){io_dir=From Processor, io_delay=0, sample_period=1, names=reg, bitwidths=32, bin_pts=0, arith_types=0, sim_port=on, show_format=on}
      mask prompts: io_dir "I/O direction"; io_delay "I/O delay"; sample_period "Sample period"; names "Bitfield names [msb...lsb]"; bitwidths "Bitfield widths"; bin_pts "Bitfield binary pts"; arith_types "Bitfield types, ufix=0, fix=1, bool=2"; sim_port "Provide sim input/output?"; show_format "Print format string?"
      mask help: A 32-bit software-accessible register. Can be divided into bitfields of varying widths and types using the fields in the block mask.
      mask init:
      | try
      |     swreg_init(gcb)
      | catch ex
      |     disp(sprintf('%s: %s', gcb, ex.message))
      |     errordlg(ex.message)
      | end
      settings: AttributesFormatString=1input:uf32.0 = 32 bits
      mask TypeOptions io_dir: To Processor | From Processor
      mask Callback io_dir:
      | mask_enables = get_param(gcb, 'MaskEnables');
      | mask_names = get_param(gcb, 'MaskNames');
      | if strcmp(get_param(gcb, 'io_dir'), 'To Processor'),
      |     mask_enables{ismember(mask_names, 'sample_period')} = 'off';
      | else
      |     mask_enables{ismember(mask_names, 'sample_period')} = 'on';
      | end
      | set_param(gcb, 'MaskEnables', mask_enables);
  rfi_convert : Subsystem  mask{shift_val=9, conv_width=9, conv_point=8}
      mask prompts: shift_val "shift"; conv_width "convert width"; conv_point "convert point"
  rfi_delay : Subsystem  mask{lat=9}
  rfi_detection0 : Subsystem  mask{din_width=18, channel_addr=9, cast_shift=5, cast_delay=1, cast_width=9, cast_point=8, post_mult_delay=0, acc_width=32, post_acc_shift=0, post_acc_width=17, post_acc_point=7, post_acc_delay=2, dout_shift=0, dout_width=18, dout_point=8, debug=1}
      mask prompts: din_width "din width"; channel_addr "channel address"; cast_shift "cast shift"; cast_delay "cast delay"; cast_width "cast width"; cast_point "cast point"; post_mult_delay "post mult delay"; acc_width "acc width"; post_acc_shift "post acc shift"; post_acc_width "post acc width"; post_acc_point "post acc point"; post_acc_delay "post acc delay"; dout_shift "dout shift"; dout_width "dout width"; dout_point "dout point"
  rfi_detection1 : Subsystem  mask{din_width=18, channel_addr=9, cast_shift=5, cast_delay=1, cast_width=9, cast_point=8, post_mult_delay=0, acc_width=32, post_acc_shift=0, post_acc_width=17, post_acc_point=7, post_acc_delay=2, dout_shift=0, dout_width=18, dout_point=8, debug=1}
      mask prompts: din_width "din width"; channel_addr "channel address"; cast_shift "cast shift"; cast_delay "cast delay"; cast_width "cast width"; cast_point "cast point"; post_mult_delay "post mult delay"; acc_width "acc width"; post_acc_shift "post acc shift"; post_acc_width "post acc width"; post_acc_point "post acc point"; post_acc_delay "post acc delay"; dout_shift "dout shift"; dout_width "dout width"; dout_point "dout point"
  rfi_detection2 : Subsystem  mask{din_width=18, channel_addr=9, cast_shift=5, cast_delay=1, cast_width=9, cast_point=8, post_mult_delay=0, acc_width=32, post_acc_shift=0, post_acc_width=17, post_acc_point=7, post_acc_delay=2, dout_shift=0, dout_width=18, dout_point=8, debug=1}
      mask prompts: din_width "din width"; channel_addr "channel address"; cast_shift "cast shift"; cast_delay "cast delay"; cast_width "cast width"; cast_point "cast point"; post_mult_delay "post mult delay"; acc_width "acc width"; post_acc_shift "post acc shift"; post_acc_width "post acc width"; post_acc_point "post acc point"; post_acc_delay "post acc delay"; dout_shift "dout shift"; dout_width "dout width"; dout_point "dout point"
  rfi_detection3 : Subsystem  mask{din_width=18, channel_addr=9, cast_shift=5, cast_delay=1, cast_width=9, cast_point=8, post_mult_delay=0, acc_width=32, post_acc_shift=0, post_acc_width=17, post_acc_point=7, post_acc_delay=2, dout_shift=0, dout_width=18, dout_point=8, debug=1}
      mask prompts: din_width "din width"; channel_addr "channel address"; cast_shift "cast shift"; cast_delay "cast delay"; cast_width "cast width"; cast_point "cast point"; post_mult_delay "post mult delay"; acc_width "acc width"; post_acc_shift "post acc shift"; post_acc_width "post acc width"; post_acc_point "post acc point"; post_acc_delay "post acc delay"; dout_shift "dout shift"; dout_width "dout width"; dout_point "dout point"
  rfi_en : Subsystem  Tag=xps:sw_reg  AncestorBlock=xps_library/software_register  mask(swreg){io_dir=From Processor, io_delay=0, sample_period=1, names=reg, bitwidths=32, bin_pts=0, arith_types=2, sim_port=on, show_format=on}
      mask prompts: io_dir "I/O direction"; io_delay "I/O delay"; sample_period "Sample period"; names "Bitfield names [msb...lsb]"; bitwidths "Bitfield widths"; bin_pts "Bitfield binary pts"; arith_types "Bitfield types, ufix=0, fix=1, bool=2"; sim_port "Provide sim input/output?"; show_format "Print format string?"
      mask help: A 32-bit software-accessible register. Can be divided into bitfields of varying widths and types using the fields in the block mask.
      mask init:
      | try
      |     swreg_init(gcb)
      | catch ex
      |     disp(sprintf('%s: %s', gcb, ex.message))
      |     errordlg(ex.message)
      | end
      settings: AttributesFormatString=1input:b = 32 bits
      mask TypeOptions io_dir: To Processor | From Processor
      mask Callback io_dir:
      | mask_enables = get_param(gcb, 'MaskEnables');
      | mask_names = get_param(gcb, 'MaskNames');
      | if strcmp(get_param(gcb, 'io_dir'), 'To Processor'),
      |     mask_enables{ismember(mask_names, 'sample_period')} = 'off';
      | else
      |     mask_enables{ismember(mask_names, 'sample_period')} = 'on';
      | end
      | set_param(gcb, 'MaskEnables', mask_enables);
  rfi_flag : Subsystem  Tag=xps:bram  AncestorBlock=xps_library/Shared_BRAM  mask{arith_type=Unsigned, addr_width=10, data_width=32, reg_prim_output=off, reg_core_output=off, optimization=Minimum_Area, data_bin_pt=0, init_vals=[0:2^10-1], sample_rate=1}
      mask prompts: arith_type "Output Data Type"; addr_width "Address width"; data_width "Data Width"; reg_prim_output "Register Primitive Output"; reg_core_output "Register Core Output"; data_bin_pt "Data Binary Point"; init_vals "Initial values (simulation only)"; sample_rate "Sample rate"
      mask init:
      | shared_bram_mask;
      mask TypeOptions arith_type: Unsigned | Signed  (2's comp)
      mask TypeOptions data_width: 8 | 16 | 32 | 64 | 128
      mask TypeOptions optimization: Minimum_Area | Low_Power
  simple_bram_vacc_0_0 : Subsystem  AncestorBlock=casper_library_accumulators/simple_bram_vacc  mask(simple_bram_vacc){vec_len=512, arith_type=Unsigned, n_bits=32, bin_pt=19}
      mask prompts: vec_len "Vector length:"; arith_type "Output type:"; n_bits "Bit width (output):"; bin_pt "Binary point (output):"
      mask help: This simple vector accumulator is based on a shift register. It outputs its previous accumulated vector after a new_acc pulse is received.
      mask init:
      | simple_bram_vacc_init(gcb, ...
      |     'vec_len', vec_len, ...
      |     'arith_type', arith_type, ...
      |     'n_bits', n_bits, ...
      |     'bin_pt', bin_pt);
      mask TypeOptions arith_type: Signed | Unsigned
  simple_bram_vacc_0_1 : Subsystem  AncestorBlock=casper_library_accumulators/simple_bram_vacc  mask(simple_bram_vacc){vec_len=512, arith_type=Unsigned, n_bits=32, bin_pt=19}
      mask prompts: vec_len "Vector length:"; arith_type "Output type:"; n_bits "Bit width (output):"; bin_pt "Binary point (output):"
      mask help: This simple vector accumulator is based on a shift register. It outputs its previous accumulated vector after a new_acc pulse is received.
      mask init:
      | simple_bram_vacc_init(gcb, ...
      |     'vec_len', vec_len, ...
      |     'arith_type', arith_type, ...
      |     'n_bits', n_bits, ...
      |     'bin_pt', bin_pt);
      mask TypeOptions arith_type: Signed | Unsigned
  simple_bram_vacc_0_10 : Subsystem  AncestorBlock=casper_library_accumulators/simple_bram_vacc  mask(simple_bram_vacc){vec_len=512, arith_type=Unsigned, n_bits=32, bin_pt=19}
      mask prompts: vec_len "Vector length:"; arith_type "Output type:"; n_bits "Bit width (output):"; bin_pt "Binary point (output):"
      mask help: This simple vector accumulator is based on a shift register. It outputs its previous accumulated vector after a new_acc pulse is received.
      mask init:
      | simple_bram_vacc_init(gcb, ...
      |     'vec_len', vec_len, ...
      |     'arith_type', arith_type, ...
      |     'n_bits', n_bits, ...
      |     'bin_pt', bin_pt);
      mask TypeOptions arith_type: Signed | Unsigned
  simple_bram_vacc_0_11 : Subsystem  AncestorBlock=casper_library_accumulators/simple_bram_vacc  mask(simple_bram_vacc){vec_len=512, arith_type=Unsigned, n_bits=32, bin_pt=19}
      mask prompts: vec_len "Vector length:"; arith_type "Output type:"; n_bits "Bit width (output):"; bin_pt "Binary point (output):"
      mask help: This simple vector accumulator is based on a shift register. It outputs its previous accumulated vector after a new_acc pulse is received.
      mask init:
      | simple_bram_vacc_init(gcb, ...
      |     'vec_len', vec_len, ...
      |     'arith_type', arith_type, ...
      |     'n_bits', n_bits, ...
      |     'bin_pt', bin_pt);
      mask TypeOptions arith_type: Signed | Unsigned
  simple_bram_vacc_0_12 : Subsystem  AncestorBlock=casper_library_accumulators/simple_bram_vacc  mask(simple_bram_vacc){vec_len=512, arith_type=Unsigned, n_bits=32, bin_pt=19}
      mask prompts: vec_len "Vector length:"; arith_type "Output type:"; n_bits "Bit width (output):"; bin_pt "Binary point (output):"
      mask help: This simple vector accumulator is based on a shift register. It outputs its previous accumulated vector after a new_acc pulse is received.
      mask init:
      | simple_bram_vacc_init(gcb, ...
      |     'vec_len', vec_len, ...
      |     'arith_type', arith_type, ...
      |     'n_bits', n_bits, ...
      |     'bin_pt', bin_pt);
      mask TypeOptions arith_type: Signed | Unsigned
  simple_bram_vacc_0_13 : Subsystem  AncestorBlock=casper_library_accumulators/simple_bram_vacc  mask(simple_bram_vacc){vec_len=512, arith_type=Unsigned, n_bits=32, bin_pt=19}
      mask prompts: vec_len "Vector length:"; arith_type "Output type:"; n_bits "Bit width (output):"; bin_pt "Binary point (output):"
      mask help: This simple vector accumulator is based on a shift register. It outputs its previous accumulated vector after a new_acc pulse is received.
      mask init:
      | simple_bram_vacc_init(gcb, ...
      |     'vec_len', vec_len, ...
      |     'arith_type', arith_type, ...
      |     'n_bits', n_bits, ...
      |     'bin_pt', bin_pt);
      mask TypeOptions arith_type: Signed | Unsigned
  simple_bram_vacc_0_14 : Subsystem  AncestorBlock=casper_library_accumulators/simple_bram_vacc  mask(simple_bram_vacc){vec_len=512, arith_type=Unsigned, n_bits=32, bin_pt=19}
      mask prompts: vec_len "Vector length:"; arith_type "Output type:"; n_bits "Bit width (output):"; bin_pt "Binary point (output):"
      mask help: This simple vector accumulator is based on a shift register. It outputs its previous accumulated vector after a new_acc pulse is received.
      mask init:
      | simple_bram_vacc_init(gcb, ...
      |     'vec_len', vec_len, ...
      |     'arith_type', arith_type, ...
      |     'n_bits', n_bits, ...
      |     'bin_pt', bin_pt);
      mask TypeOptions arith_type: Signed | Unsigned
  simple_bram_vacc_0_15 : Subsystem  AncestorBlock=casper_library_accumulators/simple_bram_vacc  mask(simple_bram_vacc){vec_len=512, arith_type=Unsigned, n_bits=32, bin_pt=19}
      mask prompts: vec_len "Vector length:"; arith_type "Output type:"; n_bits "Bit width (output):"; bin_pt "Binary point (output):"
      mask help: This simple vector accumulator is based on a shift register. It outputs its previous accumulated vector after a new_acc pulse is received.
      mask init:
      | simple_bram_vacc_init(gcb, ...
      |     'vec_len', vec_len, ...
      |     'arith_type', arith_type, ...
      |     'n_bits', n_bits, ...
      |     'bin_pt', bin_pt);
      mask TypeOptions arith_type: Signed | Unsigned
  simple_bram_vacc_0_2 : Subsystem  AncestorBlock=casper_library_accumulators/simple_bram_vacc  mask(simple_bram_vacc){vec_len=512, arith_type=Unsigned, n_bits=32, bin_pt=19}
      mask prompts: vec_len "Vector length:"; arith_type "Output type:"; n_bits "Bit width (output):"; bin_pt "Binary point (output):"
      mask help: This simple vector accumulator is based on a shift register. It outputs its previous accumulated vector after a new_acc pulse is received.
      mask init:
      | simple_bram_vacc_init(gcb, ...
      |     'vec_len', vec_len, ...
      |     'arith_type', arith_type, ...
      |     'n_bits', n_bits, ...
      |     'bin_pt', bin_pt);
      mask TypeOptions arith_type: Signed | Unsigned
  simple_bram_vacc_0_3 : Subsystem  AncestorBlock=casper_library_accumulators/simple_bram_vacc  mask(simple_bram_vacc){vec_len=512, arith_type=Unsigned, n_bits=32, bin_pt=19}
      mask prompts: vec_len "Vector length:"; arith_type "Output type:"; n_bits "Bit width (output):"; bin_pt "Binary point (output):"
      mask help: This simple vector accumulator is based on a shift register. It outputs its previous accumulated vector after a new_acc pulse is received.
      mask init:
      | simple_bram_vacc_init(gcb, ...
      |     'vec_len', vec_len, ...
      |     'arith_type', arith_type, ...
      |     'n_bits', n_bits, ...
      |     'bin_pt', bin_pt);
      mask TypeOptions arith_type: Signed | Unsigned
  simple_bram_vacc_0_4 : Subsystem  AncestorBlock=casper_library_accumulators/simple_bram_vacc  mask(simple_bram_vacc){vec_len=512, arith_type=Unsigned, n_bits=32, bin_pt=19}
      mask prompts: vec_len "Vector length:"; arith_type "Output type:"; n_bits "Bit width (output):"; bin_pt "Binary point (output):"
      mask help: This simple vector accumulator is based on a shift register. It outputs its previous accumulated vector after a new_acc pulse is received.
      mask init:
      | simple_bram_vacc_init(gcb, ...
      |     'vec_len', vec_len, ...
      |     'arith_type', arith_type, ...
      |     'n_bits', n_bits, ...
      |     'bin_pt', bin_pt);
      mask TypeOptions arith_type: Signed | Unsigned
  simple_bram_vacc_0_5 : Subsystem  AncestorBlock=casper_library_accumulators/simple_bram_vacc  mask(simple_bram_vacc){vec_len=512, arith_type=Unsigned, n_bits=32, bin_pt=19}
      mask prompts: vec_len "Vector length:"; arith_type "Output type:"; n_bits "Bit width (output):"; bin_pt "Binary point (output):"
      mask help: This simple vector accumulator is based on a shift register. It outputs its previous accumulated vector after a new_acc pulse is received.
      mask init:
      | simple_bram_vacc_init(gcb, ...
      |     'vec_len', vec_len, ...
      |     'arith_type', arith_type, ...
      |     'n_bits', n_bits, ...
      |     'bin_pt', bin_pt);
      mask TypeOptions arith_type: Signed | Unsigned
  simple_bram_vacc_0_6 : Subsystem  AncestorBlock=casper_library_accumulators/simple_bram_vacc  mask(simple_bram_vacc){vec_len=512, arith_type=Unsigned, n_bits=32, bin_pt=19}
      mask prompts: vec_len "Vector length:"; arith_type "Output type:"; n_bits "Bit width (output):"; bin_pt "Binary point (output):"
      mask help: This simple vector accumulator is based on a shift register. It outputs its previous accumulated vector after a new_acc pulse is received.
      mask init:
      | simple_bram_vacc_init(gcb, ...
      |     'vec_len', vec_len, ...
      |     'arith_type', arith_type, ...
      |     'n_bits', n_bits, ...
      |     'bin_pt', bin_pt);
      mask TypeOptions arith_type: Signed | Unsigned
  simple_bram_vacc_0_7 : Subsystem  AncestorBlock=casper_library_accumulators/simple_bram_vacc  mask(simple_bram_vacc){vec_len=512, arith_type=Unsigned, n_bits=32, bin_pt=19}
      mask prompts: vec_len "Vector length:"; arith_type "Output type:"; n_bits "Bit width (output):"; bin_pt "Binary point (output):"
      mask help: This simple vector accumulator is based on a shift register. It outputs its previous accumulated vector after a new_acc pulse is received.
      mask init:
      | simple_bram_vacc_init(gcb, ...
      |     'vec_len', vec_len, ...
      |     'arith_type', arith_type, ...
      |     'n_bits', n_bits, ...
      |     'bin_pt', bin_pt);
      mask TypeOptions arith_type: Signed | Unsigned
  simple_bram_vacc_0_8 : Subsystem  AncestorBlock=casper_library_accumulators/simple_bram_vacc  mask(simple_bram_vacc){vec_len=512, arith_type=Unsigned, n_bits=32, bin_pt=19}
      mask prompts: vec_len "Vector length:"; arith_type "Output type:"; n_bits "Bit width (output):"; bin_pt "Binary point (output):"
      mask help: This simple vector accumulator is based on a shift register. It outputs its previous accumulated vector after a new_acc pulse is received.
      mask init:
      | simple_bram_vacc_init(gcb, ...
      |     'vec_len', vec_len, ...
      |     'arith_type', arith_type, ...
      |     'n_bits', n_bits, ...
      |     'bin_pt', bin_pt);
      mask TypeOptions arith_type: Signed | Unsigned
  simple_bram_vacc_0_9 : Subsystem  AncestorBlock=casper_library_accumulators/simple_bram_vacc  mask(simple_bram_vacc){vec_len=512, arith_type=Unsigned, n_bits=32, bin_pt=19}
      mask prompts: vec_len "Vector length:"; arith_type "Output type:"; n_bits "Bit width (output):"; bin_pt "Binary point (output):"
      mask help: This simple vector accumulator is based on a shift register. It outputs its previous accumulated vector after a new_acc pulse is received.
      mask init:
      | simple_bram_vacc_init(gcb, ...
      |     'vec_len', vec_len, ...
      |     'arith_type', arith_type, ...
      |     'n_bits', n_bits, ...
      |     'bin_pt', bin_pt);
      mask TypeOptions arith_type: Signed | Unsigned
  sync_gen : Subsystem  AncestorBlock=casper_library_misc/sync_gen  mask(sync_gen){sim_acc_len=1, fft_size=4096, fft_simult_inputs=8, pfb_fir_taps=3, reorder_vec=[2,2,9], scale=1}
      mask prompts: sim_acc_len "Simulation Accumulation Length"; fft_size "FFT Size"; fft_simult_inputs "Simultaneous Inputs (FFT)"; pfb_fir_taps "Taps in pfb_fir (use 1 if no pfb_fir)"; reorder_vec "Reorder Orders (e.g. [2 2 2])"
      mask help:
      | This block computes the sync period based on system parameters as
      | described in Casper memo.  Detailed descritions of the block's
      | variables can be found in the 'Block Documentation' section of
      | the CASPER wiki.
      mask init:
      | sync_gen_init(gcb, ...
      |     'sim_acc_len', sim_acc_len, ...
      |     'fft_size', fft_size, ...
      |     'fft_simult_inputs', fft_simult_inputs,...
      |     'pfb_fir_taps', pfb_fir_taps, ...
      |     'reorder_vec', reorder_vec, ...
      |     'scale', scale);
      settings: AttributesFormatString=sim_sync_period=27648
      mask Help:
      | SyncPeriod=LCM(reorder_vec)*(acc_num)*(pfb_fir_len)*(fft_size/fft_simult_inputs)
      | 
      | See CASPER sync pulse memo for more details.
  wires:
  Black Box6/6 -> Terminator1/1
  bus_create/1(bus_out) -> pipeline276/1
  Band-Limited White Noise/1 -> asiaa_adc5g0/1(sim_a)
  Constant13/1 -> asiaa_adc5g0/3(sim_sync)
  sync_gen/1(sync_out) -> [sync_out]
  pipeline276/1 -> adcsnap0/1(din)
  Band-Limited White Noise2/1 -> asiaa_adc5g0/2(sim_c)
  asiaa_adc5g0/17(sync_out) -> Terminator/1
  asiaa_adc5g0/1(a0) -> conv_bus4/2(i0)
  asiaa_adc5g0/2(a1) -> conv_bus4/3(i1)
  asiaa_adc5g0/3(a2) -> conv_bus4/4(i2)
  asiaa_adc5g0/4(a3) -> conv_bus4/5(i3)
  asiaa_adc5g0/5(a4) -> conv_bus4/6(i4)
  asiaa_adc5g0/6(a5) -> conv_bus4/7(i5)
  asiaa_adc5g0/7(a6) -> conv_bus4/8(i6)
  asiaa_adc5g0/8(a7) -> conv_bus4/9(i7)
  bus_create1/1(bus_out) -> pipeline4/1
  pipeline4/1 -> adcsnap1/1(din)
  [cnt_rst] -> acc_cntrl0/3(rst)
  [acc_len] -> acc_cntrl0/1(acc_len)
  pipeline73/1(q) -> simple_bram_vacc_0_0/2(din)
  pre_bram_delay0/2(Out1) -> Reinterpret31/1
  pre_bram_delay0/6(valid_out) -> Counter1/2, antenna_0/3(we)
  pre_bram_delay0/1(sync_out) -> Counter1/1
  pipeline58/1(q) -> simple_bram_vacc_0_0/1(new_acc)
  pipeline60/1(q) -> simple_bram_vacc_0_1/2(din)
  pre_bram_delay0/3(Out2) -> Reinterpret24/1
  pipeline63/1(q) -> simple_bram_vacc_0_1/1(new_acc)
  pipeline64/1(q) -> simple_bram_vacc_0_2/2(din)
  pre_bram_delay0/4(Out3) -> Reinterpret25/1
  pipeline67/1(q) -> simple_bram_vacc_0_2/1(new_acc)
  pipeline68/1(q) -> simple_bram_vacc_0_3/2(din)
  pre_bram_delay0/5(Out4) -> Reinterpret26/1
  pipeline71/1(q) -> simple_bram_vacc_0_3/1(new_acc)
  Delay32/1 -> pipeline73/1(d)
  Delay34/1 -> pipeline60/1(d)
  Delay35/1 -> pipeline64/1(d)
  Delay36/1 -> pipeline68/1(d)
  acc_cntrl0/1(new_acc) -> pipeline71/1(d), pipeline67/1(d), pipeline63/1(d), pipeline58/1(d), pipeline59/1(d)
  post_fft_delay0/1(sync_out) -> pipeline72/1(d), [sync_out0]
  post_fft_delay0/2(Out1) -> [fft0_0], power16/1
  post_fft_delay0/3(Out2) -> [fft0_1], power1/1
  post_fft_delay0/4(Out3) -> power2/1, [fft0_2]
  post_fft_delay0/5(Out4) -> [fft0_3], power3/1
  Black Box1/6 -> Terminator5/1
  [cnt_rst] -> acc_cntrl1/3(rst)
  [acc_len] -> acc_cntrl1/1(acc_len)
  simple_bram_vacc_0_4/1(dout) -> pre_bram_delay1/2(In1)
  pipeline91/1(q) -> simple_bram_vacc_0_4/2(din)
  pre_bram_delay1/2(Out1) -> Reinterpret4/1
  pre_bram_delay1/6(valid_out) -> Counter2/2, antenna_1/3(we)
  pre_bram_delay1/1(sync_out) -> Counter2/1
  pipeline76/1(q) -> simple_bram_vacc_0_4/1(new_acc)
  simple_bram_vacc_0_5/1(dout) -> pre_bram_delay1/3(In2)
  pipeline78/1(q) -> simple_bram_vacc_0_5/2(din)
  pre_bram_delay1/3(Out2) -> Reinterpret1/1
  pipeline81/1(q) -> simple_bram_vacc_0_5/1(new_acc)
  simple_bram_vacc_0_6/1(dout) -> pre_bram_delay1/4(In3)
  pipeline82/1(q) -> simple_bram_vacc_0_6/2(din)
  pre_bram_delay1/4(Out3) -> Reinterpret2/1
  pipeline85/1(q) -> simple_bram_vacc_0_6/1(new_acc)
  simple_bram_vacc_0_7/1(dout) -> pre_bram_delay1/5(In4)
  simple_bram_vacc_0_7/2(valid) -> pre_bram_delay1/6(valid_in)
  pipeline86/1(q) -> simple_bram_vacc_0_7/2(din)
  pre_bram_delay1/5(Out4) -> Reinterpret3/1
  pipeline89/1(q) -> simple_bram_vacc_0_7/1(new_acc)
  Delay7/1 -> pipeline91/1(d)
  Delay8/1 -> pipeline78/1(d)
  Delay9/1 -> pipeline82/1(d)
  Delay10/1 -> pipeline86/1(d)
  acc_cntrl1/1(new_acc) -> pipeline76/1(d), pipeline89/1(d), pipeline85/1(d), pipeline81/1(d), pipeline77/1(d)
  post_fft_delay1/1(sync_out) -> [sync_out1], pipeline90/1(d)
  post_fft_delay1/2(Out1) -> power4/1, [fft1_0]
  post_fft_delay1/3(Out2) -> [fft1_1], power5/1
  post_fft_delay1/4(Out3) -> [fft1_2], power6/1
  post_fft_delay1/5(Out4) -> [fft1_3], power7/1
  asiaa_adc5g0/12(c3) -> conv_bus1/5(i3)
  asiaa_adc5g0/14(c5) -> conv_bus1/7(i5)
  asiaa_adc5g0/10(c1) -> conv_bus1/3(i1)
  asiaa_adc5g0/13(c4) -> conv_bus1/6(i4)
  asiaa_adc5g0/9(c0) -> conv_bus1/2(i0)
  asiaa_adc5g0/15(c6) -> conv_bus1/8(i6)
  asiaa_adc5g0/16(c7) -> conv_bus1/9(i7)
  asiaa_adc5g0/11(c2) -> conv_bus1/4(i2)
  Black Box2/6 -> Terminator4/1
  bus_create2/1(bus_out) -> pipeline44/1
  pipeline44/1 -> adcsnap2/1(din)
  [cnt_rst] -> acc_cntrl2/3(rst)
  [acc_len] -> acc_cntrl2/1(acc_len)
  simple_bram_vacc_0_8/1(dout) -> pre_bram_delay2/2(In1)
  pipeline104/1(q) -> simple_bram_vacc_0_8/2(din)
  pipeline50/1(q) -> pre_bram_delay2/1(sync_in)
  pipeline49/1(q) -> simple_bram_vacc_0_8/1(new_acc)
  simple_bram_vacc_0_9/1(dout) -> pre_bram_delay2/3(In2)
  pipeline52/1(q) -> simple_bram_vacc_0_9/2(din)
  pipeline55/1(q) -> simple_bram_vacc_0_9/1(new_acc)
  simple_bram_vacc_0_10/1(dout) -> pre_bram_delay2/4(In3)
  pipeline94/1(q) -> simple_bram_vacc_0_10/2(din)
  pipeline97/1(q) -> simple_bram_vacc_0_10/1(new_acc)
  simple_bram_vacc_0_11/1(dout) -> pre_bram_delay2/5(In4)
  simple_bram_vacc_0_11/2(valid) -> pre_bram_delay2/6(valid_in)
  pipeline98/1(q) -> simple_bram_vacc_0_11/2(din)
  pipeline102/1(q) -> simple_bram_vacc_0_11/1(new_acc)
  Delay43/1 -> pipeline104/1(d)
  Delay45/1 -> pipeline52/1(d)
  Delay46/1 -> pipeline94/1(d)
  Delay47/1 -> pipeline98/1(d)
  acc_cntrl2/1(new_acc) -> pipeline102/1(d), pipeline97/1(d), pipeline55/1(d), pipeline49/1(d), pipeline50/1(d)
  Black Box3/6 -> Terminator18/1
  [cnt_rst] -> acc_cntrl3/3(rst)
  [acc_len] -> acc_cntrl3/1(acc_len)
  simple_bram_vacc_0_12/1(dout) -> pre_bram_delay3/2(In1)
  pipeline123/1(q) -> simple_bram_vacc_0_12/2(din)
  pipeline108/1(q) -> pre_bram_delay3/1(sync_in)
  pre_bram_delay3/2(Out1) -> Reinterpret12/1
  pre_bram_delay3/6(valid_out) -> Counter4/2, antenna_3/3(we)
  pre_bram_delay3/1(sync_out) -> Counter4/1
  pipeline107/1(q) -> simple_bram_vacc_0_12/1(new_acc)
  simple_bram_vacc_0_13/1(dout) -> pre_bram_delay3/3(In2)
  pipeline109/1(q) -> simple_bram_vacc_0_13/2(din)
  pre_bram_delay3/3(Out2) -> Reinterpret5/1
  pipeline112/1(q) -> simple_bram_vacc_0_13/1(new_acc)
  simple_bram_vacc_0_14/1(dout) -> pre_bram_delay3/4(In3)
  pipeline113/1(q) -> simple_bram_vacc_0_14/2(din)
  pre_bram_delay3/4(Out3) -> Reinterpret6/1
  pipeline116/1(q) -> simple_bram_vacc_0_14/1(new_acc)
  simple_bram_vacc_0_15/1(dout) -> pre_bram_delay3/5(In4)
  simple_bram_vacc_0_15/2(valid) -> pre_bram_delay3/6(valid_in)
  pipeline117/1(q) -> simple_bram_vacc_0_15/2(din)
  pre_bram_delay3/5(Out4) -> Reinterpret10/1
  pipeline120/1(q) -> simple_bram_vacc_0_15/1(new_acc)
  Delay50/1 -> pipeline123/1(d)
  Delay51/1 -> pipeline109/1(d)
  Delay52/1 -> pipeline113/1(d)
  Delay1/1 -> pipeline117/1(d)
  acc_cntrl3/1(new_acc) -> pipeline108/1(d), pipeline120/1(d), pipeline116/1(d), pipeline112/1(d), pipeline107/1(d)
  power16/1 -> power_convert0/1(In1)
  power1/1 -> power_convert0/2(In2)
  power2/1 -> power_convert0/3(In3)
  power3/1 -> power_convert0/4(In4)
  pipeline72/1(q) -> pipeline127/1(d)
  power4/1 -> power_convert1/1(In1)
  power5/1 -> power_convert1/2(In2)
  power6/1 -> power_convert1/3(In3)
  power7/1 -> power_convert1/4(In4)
  power8/1 -> power_convert2/1(In1)
  power9/1 -> power_convert2/2(In2)
  power10/1 -> power_convert2/3(In3)
  power11/1 -> power_convert2/4(In4)
  power12/1 -> power_convert3/1(In1)
  power13/1 -> power_convert3/2(In2)
  power14/1 -> power_convert3/3(In3)
  power15/1 -> power_convert3/4(In4)
  pipeline90/1(q) -> pipeline128/1(d)
  pipeline103/1(q) -> pipeline129/1(d)
  pipeline122/1(q) -> pipeline130/1(d)
  Band-Limited White Noise1/1 -> asiaa_adc5g1/1(sim_a)
  Constant2/1 -> asiaa_adc5g1/3(sim_sync)
  Band-Limited White Noise3/1 -> asiaa_adc5g1/2(sim_c)
  asiaa_adc5g1/17(sync_out) -> Terminator2/1
  asiaa_adc5g1/1(a0) -> conv_bus2/2(i0)
  asiaa_adc5g1/2(a1) -> conv_bus2/3(i1)
  asiaa_adc5g1/3(a2) -> conv_bus2/4(i2)
  asiaa_adc5g1/4(a3) -> conv_bus2/5(i3)
  asiaa_adc5g1/5(a4) -> conv_bus2/6(i4)
  asiaa_adc5g1/6(a5) -> conv_bus2/7(i5)
  asiaa_adc5g1/7(a6) -> conv_bus2/8(i6)
  asiaa_adc5g1/8(a7) -> conv_bus2/9(i7)
  asiaa_adc5g1/12(c3) -> Subsystem/4(In4)
  asiaa_adc5g1/14(c5) -> Subsystem/6(In6)
  asiaa_adc5g1/10(c1) -> Subsystem/2(In2)
  asiaa_adc5g1/13(c4) -> Subsystem/5(In5)
  asiaa_adc5g1/9(c0) -> Subsystem/1(In1)
  asiaa_adc5g1/15(c6) -> Subsystem/7(In7)
  asiaa_adc5g1/16(c7) -> Subsystem/8(In8)
  asiaa_adc5g1/11(c2) -> Subsystem/3(In3)
  [sync_out] -> delay_wideband_prog0/1(sync)
  [sync_out] -> delay_wideband_prog1/1(sync)
  [sync_out] -> delay_wideband_prog2/1(sync)
  [sync_out] -> pipeline/1(d)
  [snap_trig] -> adcsnap0/2(we), adcsnap0/3(trig)
  [snap_trig] -> adcsnap1/2(we), adcsnap1/3(trig)
  [snap_trig] -> adcsnap2/2(we), adcsnap2/3(trig)
  [adc0_delay] -> delay_wideband_prog0/2(delay)
  [adc1_delay] -> delay_wideband_prog1/2(delay)
  [adc2_delay] -> delay_wideband_prog2/2(delay)
  Constant8/1 -> delay_wideband_prog0/3(ld_delay)
  Constant9/1 -> delay_wideband_prog1/3(ld_delay)
  Constant11/1 -> delay_wideband_prog2/3(ld_delay)
  delay_wideband_prog0/9(data_out7) -> pre_pfb_delay1/9(In1)
  delay_wideband_prog0/7(data_out5) -> pre_pfb_delay1/7(In8)
  delay_wideband_prog0/2(data_out0) -> pre_pfb_delay1/2(In3)
  delay_wideband_prog0/3(data_out1) -> pre_pfb_delay1/3(In4)
  delay_wideband_prog0/5(data_out3) -> pre_pfb_delay1/5(In6)
  delay_wideband_prog0/8(data_out6) -> pre_pfb_delay1/8(In9)
  delay_wideband_prog0/4(data_out2) -> pre_pfb_delay1/4(In5)
  delay_wideband_prog0/6(data_out4) -> pre_pfb_delay1/6(In7)
  delay_wideband_prog0/1(sync_out) -> pre_pfb_delay1/1(sync_in)
  delay_wideband_prog1/1(sync_out) -> pre_pfb_delay2/1(sync_in)
  delay_wideband_prog1/2(data_out0) -> pre_pfb_delay2/2(In3)
  delay_wideband_prog1/3(data_out1) -> pre_pfb_delay2/3(In4)
  delay_wideband_prog1/4(data_out2) -> pre_pfb_delay2/4(In5)
  delay_wideband_prog1/5(data_out3) -> pre_pfb_delay2/5(In6)
  delay_wideband_prog1/6(data_out4) -> pre_pfb_delay2/6(In7)
  delay_wideband_prog1/7(data_out5) -> pre_pfb_delay2/7(In8)
  delay_wideband_prog1/8(data_out6) -> pre_pfb_delay2/8(In9)
  delay_wideband_prog1/9(data_out7) -> pre_pfb_delay2/9(In1)
  delay_wideband_prog2/1(sync_out) -> pre_pfb_delay3/1(sync_in)
  delay_wideband_prog2/2(data_out0) -> pre_pfb_delay3/2(In3)
  delay_wideband_prog2/3(data_out1) -> pre_pfb_delay3/3(In4)
  delay_wideband_prog2/4(data_out2) -> pre_pfb_delay3/4(In5)
  delay_wideband_prog2/5(data_out3) -> pre_pfb_delay3/5(In6)
  delay_wideband_prog2/6(data_out4) -> pre_pfb_delay3/6(In7)
  delay_wideband_prog2/7(data_out5) -> pre_pfb_delay3/7(In8)
  delay_wideband_prog2/8(data_out6) -> pre_pfb_delay3/8(In9)
  delay_wideband_prog2/9(data_out7) -> pre_pfb_delay3/9(In1)
  conv_bus4/1(q0) -> delay_wideband_prog0/4(data_in0)
  conv_bus4/2(q1) -> delay_wideband_prog0/5(data_in1)
  conv_bus4/3(q2) -> delay_wideband_prog0/6(data_in2)
  conv_bus4/4(q3) -> delay_wideband_prog0/7(data_in3)
  conv_bus4/5(q4) -> delay_wideband_prog0/8(data_in4)
  conv_bus4/6(q5) -> delay_wideband_prog0/9(data_in5)
  conv_bus4/7(q6) -> delay_wideband_prog0/10(data_in6)
  conv_bus4/8(q7) -> delay_wideband_prog0/11(data_in7)
  conv_bus1/1(q0) -> delay_wideband_prog1/4(data_in0)
  conv_bus1/2(q1) -> delay_wideband_prog1/5(data_in1)
  conv_bus1/3(q2) -> delay_wideband_prog1/6(data_in2)
  conv_bus1/4(q3) -> delay_wideband_prog1/7(data_in3)
  conv_bus1/5(q4) -> delay_wideband_prog1/8(data_in4)
  conv_bus1/6(q5) -> delay_wideband_prog1/9(data_in5)
  conv_bus1/7(q6) -> delay_wideband_prog1/10(data_in6)
  conv_bus1/8(q7) -> delay_wideband_prog1/11(data_in7)
  conv_bus2/1(q0) -> delay_wideband_prog2/4(data_in0)
  conv_bus2/2(q1) -> delay_wideband_prog2/5(data_in1)
  conv_bus2/3(q2) -> delay_wideband_prog2/6(data_in2)
  conv_bus2/4(q3) -> delay_wideband_prog2/7(data_in3)
  conv_bus2/5(q4) -> delay_wideband_prog2/8(data_in4)
  conv_bus2/6(q5) -> delay_wideband_prog2/9(data_in5)
  conv_bus2/7(q6) -> delay_wideband_prog2/10(data_in6)
  conv_bus2/8(q7) -> delay_wideband_prog2/11(data_in7)
  pre_pfb_delay1/2(Out3) -> bus_create/1(in1), Black Box6/2
  pre_pfb_delay1/3(Out4) -> bus_create/2(in2), Black Box6/3
  pre_pfb_delay1/4(Out5) -> Black Box6/4, bus_create/3(in3)
  pre_pfb_delay1/5(Out6) -> Black Box6/5, bus_create/4(in4)
  pre_pfb_delay1/6(Out7) -> bus_create/5(in5), Black Box6/6
  pre_pfb_delay1/7(Out8) -> Black Box6/7, bus_create/6(in6)
  pre_pfb_delay1/8(Out9) -> bus_create/7(in7), Black Box6/8
  pre_pfb_delay1/9(Out1) -> Black Box6/9, bus_create/8(in8)
  pre_pfb_delay2/9(Out1) -> Black Box1/9, bus_create1/8(in8)
  pre_pfb_delay2/2(Out3) -> Black Box1/2, bus_create1/1(in1)
  pre_pfb_delay2/3(Out4) -> bus_create1/2(in2), Black Box1/3
  pre_pfb_delay2/8(Out9) -> bus_create1/7(in7), Black Box1/8
  pre_pfb_delay2/7(Out8) -> Black Box1/7, bus_create1/6(in6)
  pre_pfb_delay2/6(Out7) -> Black Box1/6, bus_create1/5(in5)
  pre_pfb_delay2/5(Out6) -> bus_create1/4(in4), Black Box1/5
  pre_pfb_delay2/4(Out5) -> Black Box1/4, bus_create1/3(in3)
  pre_pfb_delay3/9(Out1) -> Black Box2/9, bus_create2/8(in8)
  pre_pfb_delay3/8(Out9) -> Black Box2/8, bus_create2/7(in7)
  pre_pfb_delay3/7(Out8) -> bus_create2/6(in6), Black Box2/7
  pre_pfb_delay3/6(Out7) -> Black Box2/6, bus_create2/5(in5)
  pre_pfb_delay3/5(Out6) -> Black Box2/5, bus_create2/4(in4)
  pre_pfb_delay3/4(Out5) -> bus_create2/3(in3), Black Box2/4
  pre_pfb_delay3/3(Out4) -> Black Box2/3, bus_create2/2(in2)
  pre_pfb_delay3/2(Out3) -> Black Box2/2, bus_create2/1(in1)
  pipeline/1(q) -> delay_pre_pfb/1
  pre_pfb_delay1/1(sync_out) -> Black Box6/1
  pre_pfb_delay2/1(sync_out) -> Black Box1/1
  pre_pfb_delay3/1(sync_out) -> Black Box2/1
  delay_pre_pfb/1 -> Black Box3/1
  Black Box6/5 -> post_fft_delay0/5(In4)
  Black Box6/3 -> post_fft_delay0/3(In2)
  Black Box6/4 -> post_fft_delay0/4(In3)
  Black Box6/2 -> post_fft_delay0/2(In1)
  Black Box6/1 -> post_fft_delay0/1(sync_in)
  Black Box1/5 -> post_fft_delay1/5(In4)
  Black Box1/3 -> post_fft_delay1/3(In2)
  Black Box1/2 -> post_fft_delay1/2(In1)
  Black Box1/4 -> post_fft_delay1/4(In3)
  Black Box1/1 -> post_fft_delay1/1(sync_in)
  Black Box2/5 -> post_fft_delay2/5(In4)
  Black Box2/1 -> post_fft_delay2/1(sync_in)
  Black Box2/2 -> post_fft_delay2/2(In1)
  Black Box2/4 -> post_fft_delay2/4(In3)
  Black Box2/3 -> post_fft_delay2/3(In2)
  Black Box3/4 -> post_fft_delay3/4(In3)
  Black Box3/2 -> post_fft_delay3/2(In1)
  Black Box3/5 -> post_fft_delay3/5(In4)
  Black Box3/3 -> post_fft_delay3/3(In2)
  Black Box3/1 -> post_fft_delay3/1(sync_in)
  bus_create3/1(bus_out) -> pipeline6/1
  pipeline6/1 -> adcsnap3/1(din)
  [snap_trig] -> adcsnap3/2(we), adcsnap3/3(trig)
  Subsystem/8(Out8) -> bus_create3/8(in8), Black Box3/9
  Subsystem/7(Out7) -> bus_create3/7(in7), Black Box3/8
  Subsystem/6(Out6) -> bus_create3/6(in6), Black Box3/7
  Subsystem/5(Out5) -> bus_create3/5(in5), Black Box3/6
  Subsystem/4(Out4) -> bus_create3/4(in4), Black Box3/5
  Subsystem/3(Out3) -> bus_create3/3(in3), Black Box3/4
  Subsystem/2(Out2) -> bus_create3/2(in2), Black Box3/3
  Subsystem/1(Out1) -> bus_create3/1(in1), Black Box3/2
  post_fft_delay2/1(sync_out) -> [sync_out2], pipeline103/1(d)
  post_fft_delay2/2(Out1) -> power8/1, [fft2_0]
  post_fft_delay2/3(Out2) -> [fft2_1], power9/1
  post_fft_delay2/4(Out3) -> power10/1, [fft2_2]
  post_fft_delay2/5(Out4) -> power11/1, [fft2_3]
  post_fft_delay3/1(sync_out) -> [sync_out3], pipeline122/1(d)
  post_fft_delay3/2(Out1) -> power12/1, [fft3_0]
  post_fft_delay3/3(Out2) -> [fft3_1], power13/1
  post_fft_delay3/4(Out3) -> power14/1, [fft3_2]
  post_fft_delay3/5(Out4) -> [fft3_3], power15/1
  pipeline127/1(q) -> acc_cntrl0/2(sync)
  power_convert0/1(Out1) -> Delay32/1
  power_convert0/2(Out2) -> Delay34/1
  power_convert0/3(Out3) -> Delay35/1
  power_convert0/4(Out4) -> Delay36/1
  pipeline128/1(q) -> acc_cntrl1/2(sync)
  power_convert1/1(Out1) -> Delay7/1
  power_convert1/2(Out2) -> Delay8/1
  power_convert1/3(Out3) -> Delay9/1
  power_convert1/4(Out4) -> Delay10/1
  pipeline129/1(q) -> acc_cntrl2/2(sync)
  power_convert2/1(Out1) -> Delay43/1
  power_convert2/2(Out2) -> Delay45/1
  power_convert2/3(Out3) -> Delay46/1
  power_convert2/4(Out4) -> Delay47/1
  pipeline130/1(q) -> acc_cntrl3/2(sync)
  power_convert3/1(Out1) -> Delay50/1
  power_convert3/2(Out2) -> Delay51/1
  power_convert3/3(Out3) -> Delay52/1
  power_convert3/4(Out4) -> Delay1/1
  Concat/1 -> antenna_0/2(data_in)
  Counter1/1 -> antenna_0/1(addr)
  Concat1/1 -> antenna_1/2(data_in)
  Counter2/1 -> antenna_1/1(addr)
  Concat2/1 -> antenna_2/2(data_in)
  Counter3/1 -> antenna_2/1(addr)
  Concat3/1 -> antenna_3/2(data_in)
  Counter4/1 -> antenna_3/1(addr)
  simple_bram_vacc_0_0/1(dout) -> pre_bram_delay0/2(In1)
  simple_bram_vacc_0_1/1(dout) -> pre_bram_delay0/3(In2)
  simple_bram_vacc_0_2/1(dout) -> pre_bram_delay0/4(In3)
  simple_bram_vacc_0_3/1(dout) -> pre_bram_delay0/5(In4)
  simple_bram_vacc_0_3/2(valid) -> pre_bram_delay0/6(valid_in)
  pipeline59/1(q) -> pre_bram_delay0/1(sync_in)
  pipeline77/1(q) -> pre_bram_delay1/1(sync_in)
  pre_bram_delay2/1(sync_out) -> Counter3/1
  pre_bram_delay2/2(Out1) -> Reinterpret11/1
  pre_bram_delay2/3(Out2) -> Reinterpret7/1
  pre_bram_delay2/4(Out3) -> Reinterpret8/1
  pre_bram_delay2/5(Out4) -> Reinterpret9/1
  pre_bram_delay2/6(valid_out) -> Counter3/2, antenna_2/3(we)
  control/1(cnt_rst) -> [cnt_rst]
  control/2(snap_trig) -> [snap_trig]
  control/3(adc0_delay) -> [adc0_delay]
  control/4(adc1_delay) -> [adc1_delay]
  control/5(adc2_delay) -> [adc2_delay]
  control/6(adc3_delay) -> [adc3_delay]
  control/7(gbe_ip) -> [gbe_ip]
  control/8(gbe_port) -> [gbe_port]
  control/9(tge_ip) -> [tge_ip]
  control/10(tge_port) -> [tge_port]
  control/11(adc_gain) -> [adc_gain]
  control/12(rst_detection) -> [rst_detection]
  [adc_gain] -> conv_bus4/1(gain)
  [adc_gain] -> conv_bus1/1(gain)
  [adc_gain] -> conv_bus2/1(gain)
  conv_bus4/9(reduced) -> [adc0]
  conv_bus1/9(reduced) -> [adc1]
  conv_bus2/9(reduced) -> [adc2]
  [fft0_0] -> complex_add/1(ff0_ch0)
  [fft1_0] -> complex_add/2(fft1_ch0)
  [fft0_1] -> complex_add/3(fft0_ch1)
  [fft1_1] -> complex_add/4(fft1_ch1)
  [fft0_2] -> complex_add/5(fft0_ch2)
  [fft1_2] -> complex_add/6(fft1_ch2)
  [fft0_3] -> complex_add/7(fft0_ch3)
  [fft1_3] -> complex_add/8(fft1_ch3)
  [sync_out0] -> complex_add/9(sync)
  complex_add/3(ch1) -> beam_post_complex_add/3(In2)
  complex_add/1(sync_out) -> beam_post_complex_add/1(sync_in)
  complex_add/2(ch0) -> beam_post_complex_add/2(In1)
  complex_add/5(ch3) -> beam_post_complex_add/5(In4)
  complex_add/4(ch2) -> beam_post_complex_add/4(In3)
  beam_post_complex_add/5(Out4) -> concat_order/4(ch3)
  beam_post_complex_add/4(Out3) -> concat_order/3(ch2)
  beam_post_complex_add/3(Out2) -> concat_order/2(ch1)
  beam_post_complex_add/2(Out1) -> concat_order/1(ch0)
  control/13(tge_pkt) -> [tge_pkt]
  control/14(tge_sleep) -> [tge_sleep]
  control/15(tge_en) -> [tge_en]
  control/16(rst_tge) -> [tge_rst]
  beam_post_complex_add/1(sync_out) -> Black Box5/1
  concat_order/1(Out1) -> Black Box5/2
  [flag_rfi] -> Black Box5/3
  [flag_num] -> Black Box5/4
  [flag_en] -> Black Box5/5
  Black Box5/2 -> Slice2/1, Slice5/1, Slice3/1, Slice1/1
  Black Box5/1 -> Convert5/1
  control/17(flag_en) -> [flag_en]
  control/18(flag_num) -> [flag_num]
  control/19(flag_rfi) -> [flag_rfi]
  control/20(acc_len0) -> [acc_len]
  control/21(acc_len1) -> [acc_len0]
  control/22(acc_len2) -> [acc_len1]
  control/23(acc_len3) -> [acc_len2]
  control/24(acc_len4) -> [acc_len3]
  Reinterpret31/1 -> Concat/1
  Reinterpret24/1 -> Concat/2
  Reinterpret25/1 -> Concat/3
  Reinterpret26/1 -> Concat/4
  Reinterpret4/1 -> Concat1/1
  Reinterpret1/1 -> Concat1/2
  Reinterpret2/1 -> Concat1/3
  Reinterpret3/1 -> Concat1/4
  Reinterpret11/1 -> Concat2/1
  Reinterpret7/1 -> Concat2/2
  Reinterpret8/1 -> Concat2/3
  Reinterpret9/1 -> Concat2/4
  Reinterpret12/1 -> Concat3/1
  Reinterpret5/1 -> Concat3/2
  Reinterpret6/1 -> Concat3/3
  Reinterpret10/1 -> Concat3/4
  control/25(rst_dedisp) -> [rst_dedisp]
  control/26(theta1) -> [theta0]
  control/27(theta2) -> [theta1]
  control/28(theta3) -> [theta2]
  control/29(theta4) -> [theta3]
  Convert5/1 -> beam_rfi_delay/1(sync_in)
  Slice3/1 -> beam_rfi_delay/2(In1)
  Slice5/1 -> beam_rfi_delay/3(In2)
  Slice1/1 -> beam_rfi_delay/4(In3)
  Slice2/1 -> beam_rfi_delay/5(In4)
  beam_rfi_delay/2(Out1) -> beam_rfi_convert/2(In1)
  beam_rfi_delay/3(Out2) -> beam_rfi_convert/3(In2)
  beam_rfi_delay/1(sync_out) -> beam_rfi_convert/1(sync_in)
  beam_rfi_delay/4(Out3) -> beam_rfi_convert/4(In3)
  beam_rfi_delay/5(Out4) -> beam_rfi_convert/5(In4)
  beam_rfi_convert/1(sync_out) -> [beam_sync]
  beam_rfi_convert/2(Out1) -> [beam0]
  beam_rfi_convert/3(Out2) -> [beam1]
  beam_rfi_convert/4(Out3) -> [beam2]
  beam_rfi_convert/5(Out4) -> [beam3]
  rfi_delay/2(Out1) -> rfi_convert/2(In1)
  rfi_delay/3(Out2) -> rfi_convert/3(In2)
  rfi_delay/1(sync_out) -> rfi_convert/1(sync_in)
  rfi_delay/4(Out3) -> rfi_convert/4(In3)
  rfi_delay/5(Out4) -> rfi_convert/5(In4)
  [sync_out3] -> rfi_delay/1(sync_in)
  [fft3_0] -> rfi_delay/2(In1)
  [fft3_1] -> rfi_delay/3(In2)
  [fft3_2] -> rfi_delay/4(In3)
  [fft3_3] -> rfi_delay/5(In4)
  rfi_convert/1(sync_out) -> [rfi_sync]
  rfi_convert/2(Out1) -> [rfi0]
  rfi_convert/3(Out2) -> [rfi1]
  rfi_convert/4(Out3) -> [rfi2]
  rfi_convert/5(Out4) -> [rfi3]
  Reinterpret23/1 -> Concat11/1
  Reinterpret21/1 -> Concat11/2
  Reinterpret22/1 -> Concat11/3
  Reinterpret28/1 -> Concat11/4
  phase_calc/1(sync_out) -> Counter10/1
  phase_calc/2(dout_valid) -> rfi_flag/3(we), Counter10/2
  phase_calc/3(dout3) -> Reinterpret23/1
  phase_calc/4(dout2) -> Reinterpret21/1
  phase_calc/5(dout1) -> Reinterpret22/1
  phase_calc/6(dout0) -> Reinterpret28/1
  Counter10/1 -> rfi_flag/1(addr)
  Concat11/1 -> rfi_flag/2(data_in)
  c_to_ri/1 -> rfi_detection0/1(sig_re)
  c_to_ri/2 -> rfi_detection0/2(sig_im)
  c_to_ri1/1 -> rfi_detection0/3(ref_re)
  c_to_ri1/2 -> rfi_detection0/4(ref_im)
  c_to_ri2/1 -> rfi_detection1/1(sig_re)
  c_to_ri2/2 -> rfi_detection1/2(sig_im)
  c_to_ri3/1 -> rfi_detection1/3(ref_re)
  c_to_ri3/2 -> rfi_detection1/4(ref_im)
  c_to_ri4/2 -> rfi_detection2/2(sig_im)
  c_to_ri4/1 -> rfi_detection2/1(sig_re)
  c_to_ri5/2 -> rfi_detection2/4(ref_im)
  c_to_ri5/1 -> rfi_detection2/3(ref_re)
  c_to_ri6/2 -> rfi_detection3/2(sig_im)
  c_to_ri6/1 -> rfi_detection3/1(sig_re)
  c_to_ri7/1 -> rfi_detection3/3(ref_re)
  c_to_ri7/2 -> rfi_detection3/4(ref_im)
  [beam0] -> c_to_ri/1
  [rfi0] -> c_to_ri1/1
  [beam1] -> c_to_ri2/1
  [rfi1] -> c_to_ri3/1
  [beam2] -> c_to_ri4/1
  [rfi2] -> c_to_ri5/1
  [beam3] -> c_to_ri6/1
  [rfi3] -> c_to_ri7/1
  rfi_acc_len/1(in_reg) -> [rfi_acc_len]
  acc_len/1(in_reg) -> [acc_len]
  rfi_en/1(in_reg) -> [rfi_en]
  cnt_rst/1(in_reg) -> [cnt_rst]
  [rfi_acc_len] -> rfi_detection1/7(acc_len)
  [rfi_acc_len] -> rfi_detection2/7(acc_len)
  [rfi_acc_len] -> rfi_detection3/7(acc_len)
  [rfi_acc_len] -> rfi_detection0/7(acc_len)
  [cnt_rst] -> Register/2, rfi_detection0/8(cnt_rst)
  [cnt_rst] -> Register1/2, rfi_detection1/8(cnt_rst)
  [cnt_rst] -> Register2/2, rfi_detection2/8(cnt_rst)
  [cnt_rst] -> Register3/2, rfi_detection3/8(cnt_rst)
  Register/1 -> rfi_detection0/5(din_valid)
  Register1/1 -> rfi_detection1/5(din_valid)
  Register2/1 -> rfi_detection2/5(din_valid)
  Register3/1 -> rfi_detection3/5(din_valid)
  Logical/1 -> Register/3, Register/1
  [rfi_en] -> Logical/1
  [beam_sync] -> Logical/2
  [rfi_en] -> Logical1/1
  [beam_sync] -> Logical1/2
  Logical1/1 -> Register1/3, Register1/1
  [rfi_en] -> Logical2/1
  [beam_sync] -> rfi_detection2/6(sync_in), Logical2/2
  Logical2/1 -> Register2/1, Register2/3
  [rfi_en] -> Logical3/1
  [beam_sync] -> rfi_detection3/6(sync_in), Logical3/2
  Logical3/1 -> Register3/3, Register3/1
  rfi_detection3/1(pow_data) -> [rfi_pow3]
  rfi_detection3/2(corr_data) -> [rfi_corr3]
  rfi_detection2/1(pow_data) -> [rfi_pow2]
  rfi_detection2/2(corr_data) -> [rfi_corr2]
  rfi_detection1/1(pow_data) -> [rfi_pow1]
  rfi_detection1/2(corr_data) -> [rfi_corr1]
  rfi_detection0/1(pow_data) -> [rfi_pow0]
  rfi_detection0/2(corr_data) -> [rfi_corr0]
  rfi_detection3/3(dout_valid) -> [rfi_pow_valid]
  [rfi_pow_valid] -> phase_calc/2(rfi_pow_valid)
  [rfi_pow3] -> phase_calc/3(rfi_pow3)
  [rfi_corr3] -> phase_calc/4(rfi_corr3)
  [rfi_pow2] -> phase_calc/5(rfi_pow2)
  [rfi_corr2] -> phase_calc/6(rfi_corr2)
  [rfi_pow1] -> phase_calc/7(rfi_pow1)
  [rfi_corr1] -> phase_calc/8(rfi_corr1)
  [rfi_pow0] -> phase_calc/9(rfi_pow0)
  [rfi_corr0] -> phase_calc/10(rfi_corr0)
